simulink model "myo_sfun_one_myo_imu_emg"  (R2019a)
(part 8 of 12)

  "IW{2,1}(753,:)'" : Constant  Value=[0.783185612121389596040899050422012805938720703125;0.0661703247426442542344915409557870589196681976318359375;1.8359071026802709081238162980298511683940887451171875;-1.2946291113238352910030926068429835140705108642578125;-1.66363113612183166623026409070007503032684326171875;1.3769476811910852376286129583604633808135986328125;-0.82309788931886507246105111335054971277713775634765625;0.269452098677136542281829179046326316893100738525390625]
      mask Display: e = 0.06;c1 = [120 150 230]/255;c2 = ([120 150 230]+0)/383;c3 = ([120 150 230]+128)/383;patch([0 1 1 0],[0 0 1 1],c1);patch([0 1 1 1-e 1-e 0+e],[0 0 1 1-e 0+e 0+e],c2);patch([0 0 1 1-e 0+e 0+e],[0 1 1 1-e 1-e 0+e],c3);plot([0 1 1 0 0],[0 0 1 1 0]);disp('weights');
  "IW{2,1}(754,:)'" : Constant  Value=[-0.410530092885312336559167079030885361135005950927734375;-0.32543198628027558694242316050804220139980316162109375;0.257120581846906504086547329279710538685321807861328125;-1.4803527284791011542353089680545963346958160400390625;0.69265147232993451442695231889956630766391754150390625;1.1864451832958398114215015084482729434967041015625;2.49165954303533343505705488496460020542144775390625;-0.306699933021862436444138211300014518201351165771484375]
      mask Display: e = 0.06;c1 = [120 150 230]/255;c2 = ([120 150 230]+0)/383;c3 = ([120 150 230]+128)/383;patch([0 1 1 0],[0 0 1 1],c1);patch([0 1 1 1-e 1-e 0+e],[0 0 1 1-e 0+e 0+e],c2);patch([0 0 1 1-e 0+e 0+e],[0 1 1 1-e 1-e 0+e],c3);plot([0 1 1 0 0],[0 0 1 1 0]);disp('weights');
  "IW{2,1}(755,:)'" : Constant  Value=[-0.69971720416721427948658629247802309691905975341796875;0.379334814180492696511493022626382298767566680908203125;-1.66638817062355126807915439712814986705780029296875;-0.050359156796019884094750551639663171954452991485595703125;0.04393760587542960838192129813251085579395294189453125;-0.99442533329644466899566168649471364915370941162109375;-1.5735631371027520852834413744858466088771820068359375;2.045584518216794212008835529559291899204254150390625]
      mask Display: e = 0.06;c1 = [120 150 230]/255;c2 = ([120 150 230]+0)/383;c3 = ([120 150 230]+128)/383;patch([0 1 1 0],[0 0 1 1],c1);patch([0 1 1 1-e 1-e 0+e],[0 0 1 1-e 0+e 0+e],c2);patch([0 0 1 1-e 0+e 0+e],[0 1 1 1-e 1-e 0+e],c3);plot([0 1 1 0 0],[0 0 1 1 0]);disp('weights');
  "IW{2,1}(756,:)'" : Constant  Value=[1.8983314823386485681311341977561824023723602294921875;-1.6499514617594390752941535538411699235439300537109375;-1.592860658104178650518178983475081622600555419921875;-0.69510526567259212082916519648279063403606414794921875;-0.423661776374660348221112826649914495646953582763671875;0.302875746156102965134238047539838589727878570556640625;1.1171659130532229919907649673405103385448455810546875;-0.4960440878741383396999253818648867309093475341796875]
      mask Display: e = 0.06;c1 = [120 150 230]/255;c2 = ([120 150 230]+0)/383;c3 = ([120 150 230]+128)/383;patch([0 1 1 0],[0 0 1 1],c1);patch([0 1 1 1-e 1-e 0+e],[0 0 1 1-e 0+e 0+e],c2);patch([0 0 1 1-e 0+e 0+e],[0 1 1 1-e 1-e 0+e],c3);plot([0 1 1 0 0],[0 0 1 1 0]);disp('weights');
  "IW{2,1}(757,:)'" : Constant  Value=[1.5429828343096232412534618561039678752422332763671875;1.6031371671961582858756401037680916488170623779296875;0.1260080986217868292964539023159886710345745086669921875;-1.277218019145921257262443759827874600887298583984375;0.67625806402758803503871831708238460123538970947265625;0.308640418798115601095588544922065921127796173095703125;1.4325843178407087208370285225100815296173095703125;-1.352065283227812830801894961041398346424102783203125]
      mask Display: e = 0.06;c1 = [120 150 230]/255;c2 = ([120 150 230]+0)/383;c3 = ([120 150 230]+128)/383;patch([0 1 1 0],[0 0 1 1],c1);patch([0 1 1 1-e 1-e 0+e],[0 0 1 1-e 0+e 0+e],c2);patch([0 0 1 1-e 0+e 0+e],[0 1 1 1-e 1-e 0+e],c3);plot([0 1 1 0 0],[0 0 1 1 0]);disp('weights');
  "IW{2,1}(758,:)'" : Constant  Value=[-1.1493088977892480517795092964661307632923126220703125;0.198852045462145576859569473526789806783199310302734375;-0.97416051213436671840639746733359061181545257568359375;1.0286050667517485646129671295057050883769989013671875;-1.80797825924482413739724506740458309650421142578125;0.3406956718575855358466242250869981944561004638671875;1.834200275324268769594482364482246339321136474609375;-0.96161781439488447364993817245704121887683868408203125]
      mask Display: e = 0.06;c1 = [120 150 230]/255;c2 = ([120 150 230]+0)/383;c3 = ([120 150 230]+128)/383;patch([0 1 1 0],[0 0 1 1],c1);patch([0 1 1 1-e 1-e 0+e],[0 0 1 1-e 0+e 0+e],c2);patch([0 0 1 1-e 0+e 0+e],[0 1 1 1-e 1-e 0+e],c3);plot([0 1 1 0 0],[0 0 1 1 0]);disp('weights');
  "IW{2,1}(759,:)'" : Constant  Value=[1.3282172390572617448611936197266913950443267822265625;-1.6000852854439948647069513754104264080524444580078125;0.77939659454038190400382291045389138162136077880859375;1.1389255157510100868734070900245569646358489990234375;-0.0990875366675535163007992878192453645169734954833984375;1.6851010413502669482710416559712029993534088134765625;-7.354374628936846181904984920407741810777224600315093994140625e-05;1.40560043153014202488293449277989566326141357421875]
      mask Display: e = 0.06;c1 = [120 150 230]/255;c2 = ([120 150 230]+0)/383;c3 = ([120 150 230]+128)/383;patch([0 1 1 0],[0 0 1 1],c1);patch([0 1 1 1-e 1-e 0+e],[0 0 1 1-e 0+e 0+e],c2);patch([0 0 1 1-e 0+e 0+e],[0 1 1 1-e 1-e 0+e],c3);plot([0 1 1 0 0],[0 0 1 1 0]);disp('weights');
  "IW{2,1}(76,:)'" : Constant  Value=[1.5001171796290153626074470594176091253757476806640625;-1.5105423251143512697325377303059212863445281982421875;-0.1206347987803942645168575609204708598554134368896484375;1.0310345222403263232280323791201226413249969482421875;-0.47768382955221511121379762698779813945293426513671875;-1.3342813875335586271120291712577454745769500732421875;-1.6696874940304839984861473567434586584568023681640625;0.790028061013774873799775377847254276275634765625]
      mask Display: e = 0.06;c1 = [120 150 230]/255;c2 = ([120 150 230]+0)/383;c3 = ([120 150 230]+128)/383;patch([0 1 1 0],[0 0 1 1],c1);patch([0 1 1 1-e 1-e 0+e],[0 0 1 1-e 0+e 0+e],c2);patch([0 0 1 1-e 0+e 0+e],[0 1 1 1-e 1-e 0+e],c3);plot([0 1 1 0 0],[0 0 1 1 0]);disp('weights');
  "IW{2,1}(760,:)'" : Constant  Value=[-1.0176371041229881342360386042855679988861083984375;-1.872748358874109175786770720151253044605255126953125;-0.8315097219371649917007971453131176531314849853515625;0.82960320877955051610541659101727418601512908935546875;-0.7592772161929002283642375914496369659900665283203125;0.06569490608334704884185839546262286603450775146484375;1.6240039806704846814255915887770242989063262939453125;1.40670233447084580546970755676738917827606201171875]
      mask Display: e = 0.06;c1 = [120 150 230]/255;c2 = ([120 150 230]+0)/383;c3 = ([120 150 230]+128)/383;patch([0 1 1 0],[0 0 1 1],c1);patch([0 1 1 1-e 1-e 0+e],[0 0 1 1-e 0+e 0+e],c2);patch([0 0 1 1-e 0+e 0+e],[0 1 1 1-e 1-e 0+e],c3);plot([0 1 1 0 0],[0 0 1 1 0]);disp('weights');
  "IW{2,1}(761,:)'" : Constant  Value=[-1.4760895710418282522624622288276441395282745361328125;1.5449238983431639038457205970189534127712249755859375;-0.6414812240901774931245427069370634853839874267578125;1.228566998028169710011070492328144609928131103515625;-0.7253998641831866933671335573308169841766357421875;-0.477018391378114914314068073508678935468196868896484375;-1.72199388644027795436386440997011959552764892578125;0.8936550261419824447983728532562963664531707763671875]
      mask Display: e = 0.06;c1 = [120 150 230]/255;c2 = ([120 150 230]+0)/383;c3 = ([120 150 230]+128)/383;patch([0 1 1 0],[0 0 1 1],c1);patch([0 1 1 1-e 1-e 0+e],[0 0 1 1-e 0+e 0+e],c2);patch([0 0 1 1-e 0+e 0+e],[0 1 1 1-e 1-e 0+e],c3);plot([0 1 1 0 0],[0 0 1 1 0]);disp('weights');
  "IW{2,1}(762,:)'" : Constant  Value=[-1.40214953361763239314541351632215082645416259765625;0.0009893132168340671057926716258634769474156200885772705078125;-0.278198338550282586734141432316391728818416595458984375;-1.3089478916323198376403524889610707759857177734375;2.48707122269313796181222642189823091030120849609375;0.0655476063049824919648500554103520698845386505126953125;1.048706524249230387368925221380777657032012939453125;-0.61192488034971781463156048630480654537677764892578125]
      mask Display: e = 0.06;c1 = [120 150 230]/255;c2 = ([120 150 230]+0)/383;c3 = ([120 150 230]+128)/383;patch([0 1 1 0],[0 0 1 1],c1);patch([0 1 1 1-e 1-e 0+e],[0 0 1 1-e 0+e 0+e],c2);patch([0 0 1 1-e 0+e 0+e],[0 1 1 1-e 1-e 0+e],c3);plot([0 1 1 0 0],[0 0 1 1 0]);disp('weights');
  "IW{2,1}(763,:)'" : Constant  Value=[0.3202938735189400087932654059841297566890716552734375;2.180097427304347856846788999973796308040618896484375;0.6510959764016657214114047746988944709300994873046875;0.71099303337939112612531289414619095623493194580078125;2.27756408640566831991236540488898754119873046875;0.0237559841239538445389900545023920130915939807891845703125;0.12412617280098704741764237269308068789541721343994140625;0.1625160289190399065528680466741207055747509002685546875]
      mask Display: e = 0.06;c1 = [120 150 230]/255;c2 = ([120 150 230]+0)/383;c3 = ([120 150 230]+128)/383;patch([0 1 1 0],[0 0 1 1],c1);patch([0 1 1 1-e 1-e 0+e],[0 0 1 1-e 0+e 0+e],c2);patch([0 0 1 1-e 0+e 0+e],[0 1 1 1-e 1-e 0+e],c3);plot([0 1 1 0 0],[0 0 1 1 0]);disp('weights');
  "IW{2,1}(764,:)'" : Constant  Value=[-1.880922227720629447134115252993069589138031005859375;0.18169438580948515937762977046077139675617218017578125;-1.1208423860042591169161596553749404847621917724609375;0.82138794977296092358898249585763551294803619384765625;-0.445086336382885028317701880951062776148319244384765625;1.1356051656416890072165415404015220701694488525390625;1.53294095421436171733375886105932295322418212890625;1.3841953251573289040976533215143717825412750244140625]
      mask Display: e = 0.06;c1 = [120 150 230]/255;c2 = ([120 150 230]+0)/383;c3 = ([120 150 230]+128)/383;patch([0 1 1 0],[0 0 1 1],c1);patch([0 1 1 1-e 1-e 0+e],[0 0 1 1-e 0+e 0+e],c2);patch([0 0 1 1-e 0+e 0+e],[0 1 1 1-e 1-e 0+e],c3);plot([0 1 1 0 0],[0 0 1 1 0]);disp('weights');
  "IW{2,1}(765,:)'" : Constant  Value=[1.6480108777175477285936722182668745517730712890625;1.2350143728516480567947155577712692320346832275390625;-1.1626332226919344758897523206542246043682098388671875;-1.3273453269119546149568122928030788898468017578125;1.0338602880135654427107283481745980679988861083984375;0.82726662699471520401317548021324910223484039306640625;-0.868750821055978672546871166559867560863494873046875;-1.0568156825773098450582665464025922119617462158203125]
      mask Display: e = 0.06;c1 = [120 150 230]/255;c2 = ([120 150 230]+0)/383;c3 = ([120 150 230]+128)/383;patch([0 1 1 0],[0 0 1 1],c1);patch([0 1 1 1-e 1-e 0+e],[0 0 1 1-e 0+e 0+e],c2);patch([0 0 1 1-e 0+e 0+e],[0 1 1 1-e 1-e 0+e],c3);plot([0 1 1 0 0],[0 0 1 1 0]);disp('weights');
  "IW{2,1}(766,:)'" : Constant  Value=[0.2369511511416406979169124724649009294807910919189453125;-1.4120721645311677949763407013961113989353179931640625;0.37879224625033247608740794021287001669406890869140625;0.71627054433412185030505270333378575742244720458984375;-1.3351683021429676667679586898884736001491546630859375;1.5140182273159628056902192838606424629688262939453125;-1.08074438127618588367795382509939372539520263671875;1.8053836983539912619534106852370314300060272216796875]
      mask Display: e = 0.06;c1 = [120 150 230]/255;c2 = ([120 150 230]+0)/383;c3 = ([120 150 230]+128)/383;patch([0 1 1 0],[0 0 1 1],c1);patch([0 1 1 1-e 1-e 0+e],[0 0 1 1-e 0+e 0+e],c2);patch([0 0 1 1-e 0+e 0+e],[0 1 1 1-e 1-e 0+e],c3);plot([0 1 1 0 0],[0 0 1 1 0]);disp('weights');
  "IW{2,1}(767,:)'" : Constant  Value=[0.0010137896241931803990865557096867632935754954814910888671875;-1.739136278505398980342988579650409519672393798828125;0.12339190484929184188356288132126792334020137786865234375;-1.68026618448033548958164828945882618427276611328125;0.9238204519764057209840757423080503940582275390625;-0.1157783217733323322118366149879875592887401580810546875;1.4456548668953030922779134925804100930690765380859375;1.5122354198140659509164152041194029152393341064453125]
      mask Display: e = 0.06;c1 = [120 150 230]/255;c2 = ([120 150 230]+0)/383;c3 = ([120 150 230]+128)/383;patch([0 1 1 0],[0 0 1 1],c1);patch([0 1 1 1-e 1-e 0+e],[0 0 1 1-e 0+e 0+e],c2);patch([0 0 1 1-e 0+e 0+e],[0 1 1 1-e 1-e 0+e],c3);plot([0 1 1 0 0],[0 0 1 1 0]);disp('weights');
  "IW{2,1}(768,:)'" : Constant  Value=[0.57912060665102649270608026199624873697757720947265625;-0.3015274233909204237846779506071470677852630615234375;0.1761144065427179550287206666325801052153110504150390625;0.481347550919307476391395539394579827785491943359375;-0.826138806546137249853245521080680191516876220703125;2.852716196456658526159344546613283455371856689453125;-1.2339068046680565782224903159658424556255340576171875;0.0028978835039482060513538197454863620805554091930389404296875]
      mask Display: e = 0.06;c1 = [120 150 230]/255;c2 = ([120 150 230]+0)/383;c3 = ([120 150 230]+128)/383;patch([0 1 1 0],[0 0 1 1],c1);patch([0 1 1 1-e 1-e 0+e],[0 0 1 1-e 0+e 0+e],c2);patch([0 0 1 1-e 0+e 0+e],[0 1 1 1-e 1-e 0+e],c3);plot([0 1 1 0 0],[0 0 1 1 0]);disp('weights');
  "IW{2,1}(769,:)'" : Constant  Value=[0.78586784355456751338664389550103805959224700927734375;0.5155840752440845609072539446060545742511749267578125;-1.4603002716642665692603486604639329016208648681640625;-1.59285262440896335789375370950438082218170166015625;-1.46770658790118257996937245479784905910491943359375;1.213265132572129090249291039071977138519287109375;-0.98696981478665379849957162150531075894832611083984375;-1.1179206552264304708188547010649926960468292236328125]
      mask Display: e = 0.06;c1 = [120 150 230]/255;c2 = ([120 150 230]+0)/383;c3 = ([120 150 230]+128)/383;patch([0 1 1 0],[0 0 1 1],c1);patch([0 1 1 1-e 1-e 0+e],[0 0 1 1-e 0+e 0+e],c2);patch([0 0 1 1-e 0+e 0+e],[0 1 1 1-e 1-e 0+e],c3);plot([0 1 1 0 0],[0 0 1 1 0]);disp('weights');
  "IW{2,1}(77,:)'" : Constant  Value=[0.94967604944117345322496248627430759370326995849609375;-1.5403680775541050973487244846182875335216522216796875;1.5908176635751611893709878131630830466747283935546875;-0.5311955915482473589150913539924658834934234619140625;-1.1887843111091120906763762832270003855228424072265625;-1.0854926151946437951067991889431141316890716552734375;0.423786694687962650629486915931920520961284637451171875;1.466556061921565845551640450139530003070831298828125]
      mask Display: e = 0.06;c1 = [120 150 230]/255;c2 = ([120 150 230]+0)/383;c3 = ([120 150 230]+128)/383;patch([0 1 1 0],[0 0 1 1],c1);patch([0 1 1 1-e 1-e 0+e],[0 0 1 1-e 0+e 0+e],c2);patch([0 0 1 1-e 0+e 0+e],[0 1 1 1-e 1-e 0+e],c3);plot([0 1 1 0 0],[0 0 1 1 0]);disp('weights');
  "IW{2,1}(770,:)'" : Constant  Value=[-1.60309206066617715435995705774985253810882568359375;-0.51783532205714533080964656619471497833728790283203125;-1.2924390595397614589501245063729584217071533203125;-0.47354576106205537033844166217022575438022613525390625;-1.231551733349906641024062992073595523834228515625;1.282123209632743954244915585150010883808135986328125;-1.339041605027291748086781808524392545223236083984375;1.158346776423092361341105061001144349575042724609375]
      mask Display: e = 0.06;c1 = [120 150 230]/255;c2 = ([120 150 230]+0)/383;c3 = ([120 150 230]+128)/383;patch([0 1 1 0],[0 0 1 1],c1);patch([0 1 1 1-e 1-e 0+e],[0 0 1 1-e 0+e 0+e],c2);patch([0 0 1 1-e 0+e 0+e],[0 1 1 1-e 1-e 0+e],c3);plot([0 1 1 0 0],[0 0 1 1 0]);disp('weights');
  "IW{2,1}(771,:)'" : Constant  Value=[-0.10844966992756878421122479494442814029753208160400390625;-2.04097879690192485213628970086574554443359375;-1.8467790540451012315514844885910861194133758544921875;-0.304314585816960303521483410804648883640766143798828125;0.265009741844671686816781175366486422717571258544921875;0.6898099317531134477832210905035026371479034423828125;1.0382473016672901788837179992697201669216156005859375;-1.3107954550942937377300268053659237921237945556640625]
      mask Display: e = 0.06;c1 = [120 150 230]/255;c2 = ([120 150 230]+0)/383;c3 = ([120 150 230]+128)/383;patch([0 1 1 0],[0 0 1 1],c1);patch([0 1 1 1-e 1-e 0+e],[0 0 1 1-e 0+e 0+e],c2);patch([0 0 1 1-e 0+e 0+e],[0 1 1 1-e 1-e 0+e],c3);plot([0 1 1 0 0],[0 0 1 1 0]);disp('weights');
  "IW{2,1}(772,:)'" : Constant  Value=[-1.517050479000064289181182175525464117527008056640625;1.3725659899028095356499079571221955120563507080078125;1.0270065742732679137105833433452062308788299560546875;-0.93487453061604097737102847531787119805812835693359375;0.68189963435994283003083182848058640956878662109375;-1.4158641006984373778010422029183246195316314697265625;-1.5124736179747910735926552661112509667873382568359375;-0.38433165867158403106174091590219177305698394775390625]
      mask Display: e = 0.06;c1 = [120 150 230]/255;c2 = ([120 150 230]+0)/383;c3 = ([120 150 230]+128)/383;patch([0 1 1 0],[0 0 1 1],c1);patch([0 1 1 1-e 1-e 0+e],[0 0 1 1-e 0+e 0+e],c2);patch([0 0 1 1-e 0+e 0+e],[0 1 1 1-e 1-e 0+e],c3);plot([0 1 1 0 0],[0 0 1 1 0]);disp('weights');
  "IW{2,1}(773,:)'" : Constant  Value=[-1.259219760630129858469672399223782122135162353515625;0.40369571030896123087217119973502121865749359130859375;-1.45176564970109467367365141399204730987548828125;-0.590275130419540605686279377550818026065826416015625;0.6519510871785050287741114516393281519412994384765625;-1.7422522773703554843649499161983840167522430419921875;1.80382679092467324011295204400084912776947021484375;-0.337580493884244325908383643763954751193523406982421875]
      mask Display: e = 0.06;c1 = [120 150 230]/255;c2 = ([120 150 230]+0)/383;c3 = ([120 150 230]+128)/383;patch([0 1 1 0],[0 0 1 1],c1);patch([0 1 1 1-e 1-e 0+e],[0 0 1 1-e 0+e 0+e],c2);patch([0 0 1 1-e 0+e 0+e],[0 1 1 1-e 1-e 0+e],c3);plot([0 1 1 0 0],[0 0 1 1 0]);disp('weights');
  "IW{2,1}(774,:)'" : Constant  Value=[1.0494588447924539931221943334094248712062835693359375;2.2426691579786588448541806428693234920501708984375;-0.3960160180596938861441458357148803770542144775390625;-0.2418699441399993765866582862145151011645793914794921875;0.295309949651697156713936465166625566780567169189453125;0.37702138534180573703480376934749074280261993408203125;0.386653205873825289717871100947377271950244903564453125;-2.0733438359517943894161362550221383571624755859375]
      mask Display: e = 0.06;c1 = [120 150 230]/255;c2 = ([120 150 230]+0)/383;c3 = ([120 150 230]+128)/383;patch([0 1 1 0],[0 0 1 1],c1);patch([0 1 1 1-e 1-e 0+e],[0 0 1 1-e 0+e 0+e],c2);patch([0 0 1 1-e 0+e 0+e],[0 1 1 1-e 1-e 0+e],c3);plot([0 1 1 0 0],[0 0 1 1 0]);disp('weights');
  "IW{2,1}(775,:)'" : Constant  Value=[1.002703173940568515121185555472038686275482177734375;-0.454218764977076860933635771289118565618991851806640625;0.2247979254728177112010456539792357943952083587646484375;0.95350044750633167200959405818139202892780303955078125;1.497138541129345856717236529220826923847198486328125;1.8020649003205033711338955981773324310779571533203125;-0.55227649259595057440463961029308848083019256591796875;-1.7603145213687529935242537248996086418628692626953125]
      mask Display: e = 0.06;c1 = [120 150 230]/255;c2 = ([120 150 230]+0)/383;c3 = ([120 150 230]+128)/383;patch([0 1 1 0],[0 0 1 1],c1);patch([0 1 1 1-e 1-e 0+e],[0 0 1 1-e 0+e 0+e],c2);patch([0 0 1 1-e 0+e 0+e],[0 1 1 1-e 1-e 0+e],c3);plot([0 1 1 0 0],[0 0 1 1 0]);disp('weights');
  "IW{2,1}(776,:)'" : Constant  Value=[-1.22814884809633184659105609171092510223388671875;-1.0010532688682953761372118606232106685638427734375;-0.97817402122436092337665058948914520442485809326171875;-1.2737862865739355555660949903540313243865966796875;1.56447940989051659244069014675915241241455078125;1.4241609039559197658064704228308983147144317626953125;1.3307174274438879901794052784680388867855072021484375;-0.054111943261800306281816830278330598957836627960205078125]
      mask Display: e = 0.06;c1 = [120 150 230]/255;c2 = ([120 150 230]+0)/383;c3 = ([120 150 230]+128)/383;patch([0 1 1 0],[0 0 1 1],c1);patch([0 1 1 1-e 1-e 0+e],[0 0 1 1-e 0+e 0+e],c2);patch([0 0 1 1-e 0+e 0+e],[0 1 1 1-e 1-e 0+e],c3);plot([0 1 1 0 0],[0 0 1 1 0]);disp('weights');
  "IW{2,1}(777,:)'" : Constant  Value=[-1.6705477679523121903315541203483007848262786865234375;-0.50565751089381161254010521588497795164585113525390625;0.374129381175553221705598616608767770230770111083984375;1.24140950769124014385624832357279956340789794921875;1.270901094959212773716217270703054964542388916015625;1.5702246279509715076727616178686730563640594482421875;-0.66101625344364511871475542648113332688808441162109375;1.3563305258847850875980611817794851958751678466796875]
      mask Display: e = 0.06;c1 = [120 150 230]/255;c2 = ([120 150 230]+0)/383;c3 = ([120 150 230]+128)/383;patch([0 1 1 0],[0 0 1 1],c1);patch([0 1 1 1-e 1-e 0+e],[0 0 1 1-e 0+e 0+e],c2);patch([0 0 1 1-e 0+e 0+e],[0 1 1 1-e 1-e 0+e],c3);plot([0 1 1 0 0],[0 0 1 1 0]);disp('weights');
  "IW{2,1}(778,:)'" : Constant  Value=[1.35356910036644517703052770229987800121307373046875;0.477217492069804849474934371755807660520076751708984375;-1.462099461724876814372464650659821927547454833984375;0.247249741115579457773065996661898680031299591064453125;-1.157008536204823911930361646227538585662841796875;-1.55515736444071261956878515775315463542938232421875;0.451936526566375729174751540995202958583831787109375;1.6690619145797871425429548253305256366729736328125]
      mask Display: e = 0.06;c1 = [120 150 230]/255;c2 = ([120 150 230]+0)/383;c3 = ([120 150 230]+128)/383;patch([0 1 1 0],[0 0 1 1],c1);patch([0 1 1 1-e 1-e 0+e],[0 0 1 1-e 0+e 0+e],c2);patch([0 0 1 1-e 0+e 0+e],[0 1 1 1-e 1-e 0+e],c3);plot([0 1 1 0 0],[0 0 1 1 0]);disp('weights');
  "IW{2,1}(779,:)'" : Constant  Value=[-0.65572414623703323410808252447168342769145965576171875;-1.47638054734529422518107821815647184848785400390625;1.4200021275675940302107846946455538272857666015625;-0.30664106971060156592301382261211983859539031982421875;-1.170123515920813428436986214364878833293914794921875;1.0749549288145419101425659391679801046848297119140625;-1.16104467805839117744426403078250586986541748046875;-1.5631502570277360231187913086614571511745452880859375]
      mask Display: e = 0.06;c1 = [120 150 230]/255;c2 = ([120 150 230]+0)/383;c3 = ([120 150 230]+128)/383;patch([0 1 1 0],[0 0 1 1],c1);patch([0 1 1 1-e 1-e 0+e],[0 0 1 1-e 0+e 0+e],c2);patch([0 0 1 1-e 0+e 0+e],[0 1 1 1-e 1-e 0+e],c3);plot([0 1 1 0 0],[0 0 1 1 0]);disp('weights');
  "IW{2,1}(78,:)'" : Constant  Value=[-0.1407466047710739243115085628232918679714202880859375;0.73016064899796095932771322623011656105518341064453125;1.8139492608273080076486394318635575473308563232421875;-1.945663194925956407388412117143161594867706298828125;0.0617384857237628092985204375509056262671947479248046875;-0.56428916929213090991623857917147688567638397216796875;-1.5004695410340704864182725941645912826061248779296875;0.82762841741629900038645928361802361905574798583984375]
      mask Display: e = 0.06;c1 = [120 150 230]/255;c2 = ([120 150 230]+0)/383;c3 = ([120 150 230]+128)/383;patch([0 1 1 0],[0 0 1 1],c1);patch([0 1 1 1-e 1-e 0+e],[0 0 1 1-e 0+e 0+e],c2);patch([0 0 1 1-e 0+e 0+e],[0 1 1 1-e 1-e 0+e],c3);plot([0 1 1 0 0],[0 0 1 1 0]);disp('weights');
  "IW{2,1}(780,:)'" : Constant  Value=[1.20472405892639766733509532059542834758758544921875;-2.177781407949598957429770962335169315338134765625;0.879613284465513789456281301681883633136749267578125;0.5214726388915311705574140432872809469699859619140625;1.8957001374363715573423405658104456961154937744140625;-0.31560867712000117979442848081816919147968292236328125;-0.2234332478380625930380887211867957375943660736083984375;-0.193737563261967171701627421498415060341358184814453125]
      mask Display: e = 0.06;c1 = [120 150 230]/255;c2 = ([120 150 230]+0)/383;c3 = ([120 150 230]+128)/383;patch([0 1 1 0],[0 0 1 1],c1);patch([0 1 1 1-e 1-e 0+e],[0 0 1 1-e 0+e 0+e],c2);patch([0 0 1 1-e 0+e 0+e],[0 1 1 1-e 1-e 0+e],c3);plot([0 1 1 0 0],[0 0 1 1 0]);disp('weights');
  "IW{2,1}(781,:)'" : Constant  Value=[2.76122829079074971758700485224835574626922607421875;-1.0623002987083018933134326289291493594646453857421875;0.1207554539788972813862955035801860503852367401123046875;-0.307599399992625588406980341460439376533031463623046875;-0.392854501898636687684529533726163208484649658203125;0.5738833622648069621163813280873000621795654296875;-1.3719460130582936674414895605877973139286041259765625;-0.05634072474674400865524148684926331043243408203125]
      mask Display: e = 0.06;c1 = [120 150 230]/255;c2 = ([120 150 230]+0)/383;c3 = ([120 150 230]+128)/383;patch([0 1 1 0],[0 0 1 1],c1);patch([0 1 1 1-e 1-e 0+e],[0 0 1 1-e 0+e 0+e],c2);patch([0 0 1 1-e 0+e 0+e],[0 1 1 1-e 1-e 0+e],c3);plot([0 1 1 0 0],[0 0 1 1 0]);disp('weights');
  "IW{2,1}(782,:)'" : Constant  Value=[-1.9322641936651330230034773194347508251667022705078125;-1.00629887395713968345489774947054684162139892578125;1.7747060806392889187321770805283449590206146240234375;0.49385409080588671404399292441667057573795318603515625;0.7713497590596443131971682305447757244110107421875;-0.130146787075340053529970418821903876960277557373046875;1.3509523785146477781182738908682949841022491455078125;0.6259672295324729685006559520843438804149627685546875]
      mask Display: e = 0.06;c1 = [120 150 230]/255;c2 = ([120 150 230]+0)/383;c3 = ([120 150 230]+128)/383;patch([0 1 1 0],[0 0 1 1],c1);patch([0 1 1 1-e 1-e 0+e],[0 0 1 1-e 0+e 0+e],c2);patch([0 0 1 1-e 0+e 0+e],[0 1 1 1-e 1-e 0+e],c3);plot([0 1 1 0 0],[0 0 1 1 0]);disp('weights');
  "IW{2,1}(783,:)'" : Constant  Value=[1.6893988429284172436695143915130756795406341552734375;0.225913592569459253933672471248428337275981903076171875;-1.243388397209162832268702914007008075714111328125;-1.862060440104080338841185948695056140422821044921875;-0.2447434177893425266692162267645471729338169097900390625;1.3641230092016243258257190973381511867046356201171875;-0.207361012426501900574038472768734209239482879638671875;-1.0513234460344680343268919386900961399078369140625]
      mask Display: e = 0.06;c1 = [120 150 230]/255;c2 = ([120 150 230]+0)/383;c3 = ([120 150 230]+128)/383;patch([0 1 1 0],[0 0 1 1],c1);patch([0 1 1 1-e 1-e 0+e],[0 0 1 1-e 0+e 0+e],c2);patch([0 0 1 1-e 0+e 0+e],[0 1 1 1-e 1-e 0+e],c3);plot([0 1 1 0 0],[0 0 1 1 0]);disp('weights');
  "IW{2,1}(784,:)'" : Constant  Value=[1.0620272474208132251760616782121360301971435546875;0.47233971658456874731513153164996765553951263427734375;-0.172945943348280339879607936381944455206394195556640625;-1.506887071281265644273616999271325767040252685546875;1.7618509452182180563539759532432071864604949951171875;-0.5532461673119841716328437541960738599300384521484375;1.2244093360544543447332443975028581917285919189453125;-1.56237266831900978303337979014031589031219482421875]
      mask Display: e = 0.06;c1 = [120 150 230]/255;c2 = ([120 150 230]+0)/383;c3 = ([120 150 230]+128)/383;patch([0 1 1 0],[0 0 1 1],c1);patch([0 1 1 1-e 1-e 0+e],[0 0 1 1-e 0+e 0+e],c2);patch([0 0 1 1-e 0+e 0+e],[0 1 1 1-e 1-e 0+e],c3);plot([0 1 1 0 0],[0 0 1 1 0]);disp('weights');
  "IW{2,1}(785,:)'" : Constant  Value=[-0.179395783995652979836421536674606613814830780029296875;-1.6818566757074220330281377755454741418361663818359375;0.09648496457834822292998211423764587379992008209228515625;0.1518050950382008046357640296264435164630413055419921875;-0.03010888320754999403217055942150182090699672698974609375;-2.298440485049809023365696702967397868633270263671875;-1.5154241120918168217457377977552823722362518310546875;0.74505564941249524668620551892672665417194366455078125]
      mask Display: e = 0.06;c1 = [120 150 230]/255;c2 = ([120 150 230]+0)/383;c3 = ([120 150 230]+128)/383;patch([0 1 1 0],[0 0 1 1],c1);patch([0 1 1 1-e 1-e 0+e],[0 0 1 1-e 0+e 0+e],c2);patch([0 0 1 1-e 0+e 0+e],[0 1 1 1-e 1-e 0+e],c3);plot([0 1 1 0 0],[0 0 1 1 0]);disp('weights');
  "IW{2,1}(786,:)'" : Constant  Value=[-1.3425414948095168998776216540136374533176422119140625;-0.0890896214824471732729449513499275781214237213134765625;1.724918800885346659157448812038637697696685791015625;-0.10471661262302543737856552752418792806565761566162109375;0.5625814408031770685880701421410776674747467041015625;0.42245581594058012608883245775359682738780975341796875;-1.2459249951450239723982349460129626095294952392578125;-2.03035397967017150477886389126069843769073486328125]
      mask Display: e = 0.06;c1 = [120 150 230]/255;c2 = ([120 150 230]+0)/383;c3 = ([120 150 230]+128)/383;patch([0 1 1 0],[0 0 1 1],c1);patch([0 1 1 1-e 1-e 0+e],[0 0 1 1-e 0+e 0+e],c2);patch([0 0 1 1-e 0+e 0+e],[0 1 1 1-e 1-e 0+e],c3);plot([0 1 1 0 0],[0 0 1 1 0]);disp('weights');
  "IW{2,1}(787,:)'" : Constant  Value=[1.0854688131216720936578212786116637289524078369140625;1.786746059171278933064286320586688816547393798828125;0.12200539984674622917548703071588533930480480194091796875;-0.81146003915904285630489312097779475152492523193359375;0.5279805453242392143664574177819304168224334716796875;0.90394730071178852615076948495698161423206329345703125;-1.448571074143185644089726338279433548450469970703125;-1.6602820646698066564539431055891327559947967529296875]
      mask Display: e = 0.06;c1 = [120 150 230]/255;c2 = ([120 150 230]+0)/383;c3 = ([120 150 230]+128)/383;patch([0 1 1 0],[0 0 1 1],c1);patch([0 1 1 1-e 1-e 0+e],[0 0 1 1-e 0+e 0+e],c2);patch([0 0 1 1-e 0+e 0+e],[0 1 1 1-e 1-e 0+e],c3);plot([0 1 1 0 0],[0 0 1 1 0]);disp('weights');
  "IW{2,1}(788,:)'" : Constant  Value=[-0.4698990953664019531998974343878217041492462158203125;2.228625086753846407106038896017707884311676025390625;0.97039922697363512060775292411562986671924591064453125;1.18753777081516975755448584095574915409088134765625;-1.2771933791042002770410590528626926243305206298828125;-0.19264632613096621671644470552564598619937896728515625;-0.6946821823975983800636413434403948485851287841796875;-1.1048478483617836243269039186998270452022552490234375]
      mask Display: e = 0.06;c1 = [120 150 230]/255;c2 = ([120 150 230]+0)/383;c3 = ([120 150 230]+128)/383;patch([0 1 1 0],[0 0 1 1],c1);patch([0 1 1 1-e 1-e 0+e],[0 0 1 1-e 0+e 0+e],c2);patch([0 0 1 1-e 0+e 0+e],[0 1 1 1-e 1-e 0+e],c3);plot([0 1 1 0 0],[0 0 1 1 0]);disp('weights');
  "IW{2,1}(789,:)'" : Constant  Value=[-1.1954349322313342351975506971939466893672943115234375;0.254954615905215342674949852153076790273189544677734375;-0.729027390173369926884561209590174257755279541015625;-1.2801448826580050788237485903664492070674896240234375;1.7653475584719651170217957769636996090412139892578125;1.273154332788164477818781961104832589626312255859375;0.297162851983625297958013788957032375037670135498046875;1.607461357218479491848484030924737453460693359375]
      mask Display: e = 0.06;c1 = [120 150 230]/255;c2 = ([120 150 230]+0)/383;c3 = ([120 150 230]+128)/383;patch([0 1 1 0],[0 0 1 1],c1);patch([0 1 1 1-e 1-e 0+e],[0 0 1 1-e 0+e 0+e],c2);patch([0 0 1 1-e 0+e 0+e],[0 1 1 1-e 1-e 0+e],c3);plot([0 1 1 0 0],[0 0 1 1 0]);disp('weights');
  "IW{2,1}(79,:)'" : Constant  Value=[-1.454345653793586823354644366190768778324127197265625;-1.5000053456295894260819068222190253436565399169921875;-0.1190879144108819287506406681131920777261257171630859375;0.01259612237224565743642923365541719249449670314788818359375;1.4220388141981465945917761928285472095012664794921875;-0.350444949810018446800796709794667549431324005126953125;-1.4862134480305819739243133881245739758014678955078125;1.6082221761231014767190572456456720829010009765625]
      mask Display: e = 0.06;c1 = [120 150 230]/255;c2 = ([120 150 230]+0)/383;c3 = ([120 150 230]+128)/383;patch([0 1 1 0],[0 0 1 1],c1);patch([0 1 1 1-e 1-e 0+e],[0 0 1 1-e 0+e 0+e],c2);patch([0 0 1 1-e 0+e 0+e],[0 1 1 1-e 1-e 0+e],c3);plot([0 1 1 0 0],[0 0 1 1 0]);disp('weights');
  "IW{2,1}(790,:)'" : Constant  Value=[-0.3499584335750405283960162705625407397747039794921875;1.4123167729368490963537396964966319501399993896484375;1.0513137201449305191403027492924593389034271240234375;-1.6753309471439685740534741853480227291584014892578125;-0.143085928295401398901987022327375598251819610595703125;0.9409164128731362097823875956237316131591796875;-1.2519447014244640126179319850052706897258758544921875;-1.66698599786439505265889238216914236545562744140625]
      mask Display: e = 0.06;c1 = [120 150 230]/255;c2 = ([120 150 230]+0)/383;c3 = ([120 150 230]+128)/383;patch([0 1 1 0],[0 0 1 1],c1);patch([0 1 1 1-e 1-e 0+e],[0 0 1 1-e 0+e 0+e],c2);patch([0 0 1 1-e 0+e 0+e],[0 1 1 1-e 1-e 0+e],c3);plot([0 1 1 0 0],[0 0 1 1 0]);disp('weights');
  "IW{2,1}(791,:)'" : Constant  Value=[-1.6212226087080814362906266978825442492961883544921875;-0.00664598725078462647386512429648064426146447658538818359375;-0.497774706925136645185858697004732675850391387939453125;-0.8965190674538294768325386030483059585094451904296875;1.8128340585994402456293528302921913564205169677734375;-0.251152548948948839413475297988043166697025299072265625;0.11213514945235657227495806864681071601808071136474609375;-1.9991787235258726695974473841488361358642578125]
      mask Display: e = 0.06;c1 = [120 150 230]/255;c2 = ([120 150 230]+0)/383;c3 = ([120 150 230]+128)/383;patch([0 1 1 0],[0 0 1 1],c1);patch([0 1 1 1-e 1-e 0+e],[0 0 1 1-e 0+e 0+e],c2);patch([0 0 1 1-e 0+e 0+e],[0 1 1 1-e 1-e 0+e],c3);plot([0 1 1 0 0],[0 0 1 1 0]);disp('weights');
  "IW{2,1}(792,:)'" : Constant  Value=[-1.6602606604656544586617883396684192121028900146484375;-0.8496114760869364346262955223210155963897705078125;-0.35104782957804758769526642936398275196552276611328125;-1.656826004383271655484577422612346708774566650390625;-1.4346878897252810514117982165771536529064178466796875;0.165466029757858124060732052384992130100727081298828125;1.5734664279879722048605117379338480532169342041015625;0.337872835146016570195826034250785596668720245361328125]
      mask Display: e = 0.06;c1 = [120 150 230]/255;c2 = ([120 150 230]+0)/383;c3 = ([120 150 230]+128)/383;patch([0 1 1 0],[0 0 1 1],c1);patch([0 1 1 1-e 1-e 0+e],[0 0 1 1-e 0+e 0+e],c2);patch([0 0 1 1-e 0+e 0+e],[0 1 1 1-e 1-e 0+e],c3);plot([0 1 1 0 0],[0 0 1 1 0]);disp('weights');
  "IW{2,1}(793,:)'" : Constant  Value=[0.1354401986727943596466872122618951834738254547119140625;1.4280561271352458785344197167432866990566253662109375;-1.87261754727813212184628355316817760467529296875;-0.94910855722564801961738112368038855493068695068359375;-1.1031033185725658274378702117246575653553009033203125;-0.0222369875416463837203284725774210528470575809478759765625;-0.1605962650882052089595930510768084786832332611083984375;-1.7818971070551381519209144244086928665637969970703125]
      mask Display: e = 0.06;c1 = [120 150 230]/255;c2 = ([120 150 230]+0)/383;c3 = ([120 150 230]+128)/383;patch([0 1 1 0],[0 0 1 1],c1);patch([0 1 1 1-e 1-e 0+e],[0 0 1 1-e 0+e 0+e],c2);patch([0 0 1 1-e 0+e 0+e],[0 1 1 1-e 1-e 0+e],c3);plot([0 1 1 0 0],[0 0 1 1 0]);disp('weights');
  "IW{2,1}(794,:)'" : Constant  Value=[-0.0960306740130501823582420684033422730863094329833984375;0.8638031410457929215596095673390664160251617431640625;-1.96871235086645501866087215603329241275787353515625;1.7314153981485873590173696356941945850849151611328125;0.1530734069582344869520085239855688996613025665283203125;-0.440234092943701416089652411756105720996856689453125;1.1041120436467135590419275104068219661712646484375;-1.3741051332568099407893669194891117513179779052734375]
      mask Display: e = 0.06;c1 = [120 150 230]/255;c2 = ([120 150 230]+0)/383;c3 = ([120 150 230]+128)/383;patch([0 1 1 0],[0 0 1 1],c1);patch([0 1 1 1-e 1-e 0+e],[0 0 1 1-e 0+e 0+e],c2);patch([0 0 1 1-e 0+e 0+e],[0 1 1 1-e 1-e 0+e],c3);plot([0 1 1 0 0],[0 0 1 1 0]);disp('weights');
  "IW{2,1}(795,:)'" : Constant  Value=[-1.74714618328577131478596129454672336578369140625;1.4846747087115963470438373406068421900272369384765625;1.07823301920891623240095213986933231353759765625;-1.379851251816174961817296207300387322902679443359375;0.069145191657301430243620643523172475397586822509765625;-0.9033876654740475853344605638994835317134857177734375;-1.3328426873114216366644768640981055796146392822265625;-0.311923707529923321946085934541770257055759429931640625]
      mask Display: e = 0.06;c1 = [120 150 230]/255;c2 = ([120 150 230]+0)/383;c3 = ([120 150 230]+128)/383;patch([0 1 1 0],[0 0 1 1],c1);patch([0 1 1 1-e 1-e 0+e],[0 0 1 1-e 0+e 0+e],c2);patch([0 0 1 1-e 0+e 0+e],[0 1 1 1-e 1-e 0+e],c3);plot([0 1 1 0 0],[0 0 1 1 0]);disp('weights');
  "IW{2,1}(796,:)'" : Constant  Value=[1.5360295984492624565831420113681815564632415771484375;-1.7131536346822178185078655587858520448207855224609375;1.5768894968390656519119374934234656393527984619140625;0.173944353712400745504140786579228006303310394287109375;0.79084525076776934771061178253148682415485382080078125;-1.5519147608880408117926208433345891535282135009765625;0.449312404307729895691636556875891983509063720703125;0.2008602463838435603360466075173462741076946258544921875]
      mask Display: e = 0.06;c1 = [120 150 230]/255;c2 = ([120 150 230]+0)/383;c3 = ([120 150 230]+128)/383;patch([0 1 1 0],[0 0 1 1],c1);patch([0 1 1 1-e 1-e 0+e],[0 0 1 1-e 0+e 0+e],c2);patch([0 0 1 1-e 0+e 0+e],[0 1 1 1-e 1-e 0+e],c3);plot([0 1 1 0 0],[0 0 1 1 0]);disp('weights');
  "IW{2,1}(797,:)'" : Constant  Value=[-1.495008703605724686980238402611576020717620849609375;1.9677376501445831280534548568539321422576904296875;-0.8889135426196619338412574506946839392185211181640625;-0.68873017130275016040030777730862610042095184326171875;0.01846611302918534092132318846779526211321353912353515625;-0.90698722045707336203435033894493244588375091552734375;0.386944048199925505482354992636828683316707611083984375;-1.628627614236950904569312115199863910675048828125]
      mask Display: e = 0.06;c1 = [120 150 230]/255;c2 = ([120 150 230]+0)/383;c3 = ([120 150 230]+128)/383;patch([0 1 1 0],[0 0 1 1],c1);patch([0 1 1 1-e 1-e 0+e],[0 0 1 1-e 0+e 0+e],c2);patch([0 0 1 1-e 0+e 0+e],[0 1 1 1-e 1-e 0+e],c3);plot([0 1 1 0 0],[0 0 1 1 0]);disp('weights');
  "IW{2,1}(798,:)'" : Constant  Value=[1.596004342975323897491080060717649757862091064453125;0.0640950793087518289059545395502937026321887969970703125;0.6741903079137110399443599817459471523761749267578125;0.48545664911829355947503472634707577526569366455078125;1.4778553222691892532481006128364242613315582275390625;-1.9975412567322836654426509994664229452610015869140625;-0.273894928528651104837621232945821247994899749755859375;-1.2236279018843436716679207165725529193878173828125]
      mask Display: e = 0.06;c1 = [120 150 230]/255;c2 = ([120 150 230]+0)/383;c3 = ([120 150 230]+128)/383;patch([0 1 1 0],[0 0 1 1],c1);patch([0 1 1 1-e 1-e 0+e],[0 0 1 1-e 0+e 0+e],c2);patch([0 0 1 1-e 0+e 0+e],[0 1 1 1-e 1-e 0+e],c3);plot([0 1 1 0 0],[0 0 1 1 0]);disp('weights');
  "IW{2,1}(799,:)'" : Constant  Value=[1.4770375632864567450042159180156886577606201171875;0.693385839689065530677680726512335240840911865234375;-0.71747562482047311238630982188624329864978790283203125;0.5514079574493659929856903545442037284374237060546875;1.537506493843416865985318509046919643878936767578125;0.79357515376455667333033261456876061856746673583984375;-1.76544500847806862253719373256899416446685791015625;1.1878881439392756647066562436521053314208984375]
      mask Display: e = 0.06;c1 = [120 150 230]/255;c2 = ([120 150 230]+0)/383;c3 = ([120 150 230]+128)/383;patch([0 1 1 0],[0 0 1 1],c1);patch([0 1 1 1-e 1-e 0+e],[0 0 1 1-e 0+e 0+e],c2);patch([0 0 1 1-e 0+e 0+e],[0 1 1 1-e 1-e 0+e],c3);plot([0 1 1 0 0],[0 0 1 1 0]);disp('weights');
  "IW{2,1}(8,:)'" : Constant  Value=[1.6190915800654364087307612862787209451198577880859375;-1.002926456833790336276024390826933085918426513671875;-1.343600877266364790330044343136250972747802734375;0.92353566004879483752887381342588923871517181396484375;-1.18433082284919510840381917660124599933624267578125;0.317507488243029711849629848074982874095439910888671875;-1.7946898445228784968463742188760079443454742431640625;-0.0787404021836220768815195469869649969041347503662109375]
      mask Display: e = 0.06;c1 = [120 150 230]/255;c2 = ([120 150 230]+0)/383;c3 = ([120 150 230]+128)/383;patch([0 1 1 0],[0 0 1 1],c1);patch([0 1 1 1-e 1-e 0+e],[0 0 1 1-e 0+e 0+e],c2);patch([0 0 1 1-e 0+e 0+e],[0 1 1 1-e 1-e 0+e],c3);plot([0 1 1 0 0],[0 0 1 1 0]);disp('weights');
  "IW{2,1}(80,:)'" : Constant  Value=[0.9478079839795459093920726445503532886505126953125;-0.31673347780162064424303025589324533939361572265625;-1.890888192690478586399649429949931800365447998046875;1.2749156898670095383607758776634000241756439208984375;0.09402725139458263658998049550064024515450000762939453125;-1.5645932256938752669128689376520924270153045654296875;0.07943804668258443169026605801263940520584583282470703125;-1.53590401401625431532238508225418627262115478515625]
      mask Display: e = 0.06;c1 = [120 150 230]/255;c2 = ([120 150 230]+0)/383;c3 = ([120 150 230]+128)/383;patch([0 1 1 0],[0 0 1 1],c1);patch([0 1 1 1-e 1-e 0+e],[0 0 1 1-e 0+e 0+e],c2);patch([0 0 1 1-e 0+e 0+e],[0 1 1 1-e 1-e 0+e],c3);plot([0 1 1 0 0],[0 0 1 1 0]);disp('weights');
  "IW{2,1}(800,:)'" : Constant  Value=[1.5695590533465229032827892297063954174518585205078125;1.0744248492502819214422515869955532252788543701171875;0.6560393990154651522317408307571895420551300048828125;1.74659960593104113257822973537258803844451904296875;-0.74321026821185787181178739047027193009853363037109375;-0.09591821726676737214223322780526359565556049346923828125;1.3464183066128418975182512440369464457035064697265625;1.248659653235780542246402546879835426807403564453125]
      mask Display: e = 0.06;c1 = [120 150 230]/255;c2 = ([120 150 230]+0)/383;c3 = ([120 150 230]+128)/383;patch([0 1 1 0],[0 0 1 1],c1);patch([0 1 1 1-e 1-e 0+e],[0 0 1 1-e 0+e 0+e],c2);patch([0 0 1 1-e 0+e 0+e],[0 1 1 1-e 1-e 0+e],c3);plot([0 1 1 0 0],[0 0 1 1 0]);disp('weights');
  "IW{2,1}(801,:)'" : Constant  Value=[2.0798246771491175621804359252564609050750732421875;1.4660222130354785274874984679627232253551483154296875;0.793556890082757870885643569636158645153045654296875;0.341211262274816296002910576135036535561084747314453125;0.1464014518007050458248130553329247049987316131591796875;-0.312854385738075502221278156866901554167270660400390625;-1.4814224546802143844814736439730040729045867919921875;1.21354857077294919776022652513347566127777099609375]
      mask Display: e = 0.06;c1 = [120 150 230]/255;c2 = ([120 150 230]+0)/383;c3 = ([120 150 230]+128)/383;patch([0 1 1 0],[0 0 1 1],c1);patch([0 1 1 1-e 1-e 0+e],[0 0 1 1-e 0+e 0+e],c2);patch([0 0 1 1-e 0+e 0+e],[0 1 1 1-e 1-e 0+e],c3);plot([0 1 1 0 0],[0 0 1 1 0]);disp('weights');
  "IW{2,1}(802,:)'" : Constant  Value=[-0.291074389229205976459269322731415741145610809326171875;1.9132814454774391688118839738308452069759368896484375;0.09552870719985724623501965879768249578773975372314453125;-1.8663400259594682406572019317536614835262298583984375;-1.19725755615584450453070530784316360950469970703125;0.43867878643791391457540385090396739542484283447265625;-1.38617905284088482886772908386774361133575439453125;0.519357788722857538488142381538636982440948486328125]
      mask Display: e = 0.06;c1 = [120 150 230]/255;c2 = ([120 150 230]+0)/383;c3 = ([120 150 230]+128)/383;patch([0 1 1 0],[0 0 1 1],c1);patch([0 1 1 1-e 1-e 0+e],[0 0 1 1-e 0+e 0+e],c2);patch([0 0 1 1-e 0+e 0+e],[0 1 1 1-e 1-e 0+e],c3);plot([0 1 1 0 0],[0 0 1 1 0]);disp('weights');
  "IW{2,1}(803,:)'" : Constant  Value=[1.5759999811541558489835779255372472107410430908203125;-1.33066715101493660000642194063402712345123291015625;1.0661567719787232721984082672861404716968536376953125;1.0488956736169534611491371833835728466510772705078125;0.8921151973905649956719798865378834307193756103515625;1.26977347895268533051194026484154164791107177734375;1.4620069653833793754671432907343842089176177978515625;-0.00697567377681724935800655629236644017510116100311279296875]
      mask Display: e = 0.06;c1 = [120 150 230]/255;c2 = ([120 150 230]+0)/383;c3 = ([120 150 230]+128)/383;patch([0 1 1 0],[0 0 1 1],c1);patch([0 1 1 1-e 1-e 0+e],[0 0 1 1-e 0+e 0+e],c2);patch([0 0 1 1-e 0+e 0+e],[0 1 1 1-e 1-e 0+e],c3);plot([0 1 1 0 0],[0 0 1 1 0]);disp('weights');
  "IW{2,1}(804,:)'" : Constant  Value=[-1.5331632006206203922005215645185671746730804443359375;1.616423670938370804606165620498359203338623046875;-0.269097413861498380160952592632384039461612701416015625;-1.6522077961869083839729910323512740433216094970703125;1.406510001697613976290313075878657400608062744140625;-0.5918798046138886714828686308464966714382171630859375;-0.2071267000531098745330638166706194169819355010986328125;-0.9428369908205571636727881923434324562549591064453125]
      mask Display: e = 0.06;c1 = [120 150 230]/255;c2 = ([120 150 230]+0)/383;c3 = ([120 150 230]+128)/383;patch([0 1 1 0],[0 0 1 1],c1);patch([0 1 1 1-e 1-e 0+e],[0 0 1 1-e 0+e 0+e],c2);patch([0 0 1 1-e 0+e 0+e],[0 1 1 1-e 1-e 0+e],c3);plot([0 1 1 0 0],[0 0 1 1 0]);disp('weights');
  "IW{2,1}(805,:)'" : Constant  Value=[-1.8466700241231401857788796405657194554805755615234375;-1.106214529640654919973030700930394232273101806640625;-0.58093306234666719500836506995256058871746063232421875;-0.06168916802374783958651249804461258463561534881591796875;1.5031577493678833779000569847994484007358551025390625;-0.807364994751129216865592752583324909210205078125;-1.7622619695567645070610751645290292799472808837890625;-0.15228251029610639921685333320056088268756866455078125]
      mask Display: e = 0.06;c1 = [120 150 230]/255;c2 = ([120 150 230]+0)/383;c3 = ([120 150 230]+128)/383;patch([0 1 1 0],[0 0 1 1],c1);patch([0 1 1 1-e 1-e 0+e],[0 0 1 1-e 0+e 0+e],c2);patch([0 0 1 1-e 0+e 0+e],[0 1 1 1-e 1-e 0+e],c3);plot([0 1 1 0 0],[0 0 1 1 0]);disp('weights');
  "IW{2,1}(806,:)'" : Constant  Value=[-1.47822875434379152892461206647567451000213623046875;0.72736327466593586610343891152297146618366241455078125;1.31279981257430922170215126243419945240020751953125;-1.275088111978301963489457193645648658275604248046875;-0.429694499564222731624596463007037527859210968017578125;-1.1487674103736242869899797369726002216339111328125;1.5976098856980593954091318664723075926303863525390625;0.96328808893617201558612350709154270589351654052734375]
      mask Display: e = 0.06;c1 = [120 150 230]/255;c2 = ([120 150 230]+0)/383;c3 = ([120 150 230]+128)/383;patch([0 1 1 0],[0 0 1 1],c1);patch([0 1 1 1-e 1-e 0+e],[0 0 1 1-e 0+e 0+e],c2);patch([0 0 1 1-e 0+e 0+e],[0 1 1 1-e 1-e 0+e],c3);plot([0 1 1 0 0],[0 0 1 1 0]);disp('weights');
  "IW{2,1}(807,:)'" : Constant  Value=[0.315727944716246378131785377263440750539302825927734375;0.93650927809922779321283314857282675802707672119140625;-0.77464419006669604783610338927246630191802978515625;2.129639260131461764302684969152323901653289794921875;1.698699787103432612411779700778424739837646484375;-0.1245995104072742665213269219748326577246189117431640625;-1.39309590516954973082874857936985790729522705078125;-0.283222079422675798721087403464480303227901458740234375]
      mask Display: e = 0.06;c1 = [120 150 230]/255;c2 = ([120 150 230]+0)/383;c3 = ([120 150 230]+128)/383;patch([0 1 1 0],[0 0 1 1],c1);patch([0 1 1 1-e 1-e 0+e],[0 0 1 1-e 0+e 0+e],c2);patch([0 0 1 1-e 0+e 0+e],[0 1 1 1-e 1-e 0+e],c3);plot([0 1 1 0 0],[0 0 1 1 0]);disp('weights');
  "IW{2,1}(808,:)'" : Constant  Value=[-1.5618555574041301792220792776788584887981414794921875;-1.4015706717236182665686783366254530847072601318359375;-0.9671759623680686868141265222220681607723236083984375;-1.5653136004638257272603141245781444013118743896484375;0.519447335598108406173878393019549548625946044921875;1.3042526563493572755447758027003146708011627197265625;1.032454056462201119614974231808446347713470458984375;-0.447304036868745036326089348222012631595134735107421875]
      mask Display: e = 0.06;c1 = [120 150 230]/255;c2 = ([120 150 230]+0)/383;c3 = ([120 150 230]+128)/383;patch([0 1 1 0],[0 0 1 1],c1);patch([0 1 1 1-e 1-e 0+e],[0 0 1 1-e 0+e 0+e],c2);patch([0 0 1 1-e 0+e 0+e],[0 1 1 1-e 1-e 0+e],c3);plot([0 1 1 0 0],[0 0 1 1 0]);disp('weights');
  "IW{2,1}(809,:)'" : Constant  Value=[-0.64061148040321558294607484640437178313732147216796875;0.455821452798865822675367098781862296164035797119140625;1.6715871099535071220287818505312316119670867919921875;-1.2786896327983845456088829450891353189945220947265625;-1.1969343266811931503212917959899641573429107666015625;-0.06553992843245314003919332890291116200387477874755859375;-1.63799050658778444500285331741906702518463134765625;-1.3579867239216465435447389609180390834808349609375]
      mask Display: e = 0.06;c1 = [120 150 230]/255;c2 = ([120 150 230]+0)/383;c3 = ([120 150 230]+128)/383;patch([0 1 1 0],[0 0 1 1],c1);patch([0 1 1 1-e 1-e 0+e],[0 0 1 1-e 0+e 0+e],c2);patch([0 0 1 1-e 0+e 0+e],[0 1 1 1-e 1-e 0+e],c3);plot([0 1 1 0 0],[0 0 1 1 0]);disp('weights');
  "IW{2,1}(81,:)'" : Constant  Value=[-1.26832215508676693360712306457571685314178466796875;-0.409981797206467379890426627753186039626598358154296875;-1.361928641123699268433711040415801107883453369140625;0.99313946280979947811573538274387829005718231201171875;0.426757083082677179941555323239299468696117401123046875;1.471937926405171737087584915570914745330810546875;-1.58385752210059127520480615203268826007843017578125;-1.3353107390260685605198887060396373271942138671875]
      mask Display: e = 0.06;c1 = [120 150 230]/255;c2 = ([120 150 230]+0)/383;c3 = ([120 150 230]+128)/383;patch([0 1 1 0],[0 0 1 1],c1);patch([0 1 1 1-e 1-e 0+e],[0 0 1 1-e 0+e 0+e],c2);patch([0 0 1 1-e 0+e 0+e],[0 1 1 1-e 1-e 0+e],c3);plot([0 1 1 0 0],[0 0 1 1 0]);disp('weights');
  "IW{2,1}(810,:)'" : Constant  Value=[0.87325255156883685447866128015448339283466339111328125;0.63010602895520351207636622348218224942684173583984375;1.719254592818991955738283650134690105915069580078125;0.0264765265887349186824106794801991782151162624359130859375;2.00842846918101169961801133467815816402435302734375;-0.9021620153238962824815416752244345843791961669921875;-1.2818497011301801524751908800681121647357940673828125;-0.64689828158795326107366463475045748054981231689453125]
      mask Display: e = 0.06;c1 = [120 150 230]/255;c2 = ([120 150 230]+0)/383;c3 = ([120 150 230]+128)/383;patch([0 1 1 0],[0 0 1 1],c1);patch([0 1 1 1-e 1-e 0+e],[0 0 1 1-e 0+e 0+e],c2);patch([0 0 1 1-e 0+e 0+e],[0 1 1 1-e 1-e 0+e],c3);plot([0 1 1 0 0],[0 0 1 1 0]);disp('weights');
  "IW{2,1}(811,:)'" : Constant  Value=[-1.212607417873442727795918472111225128173828125;0.23395862819571722202027785897371359169483184814453125;0.7128154408211326842348398713511414825916290283203125;1.6932202821937440972988042631186544895172119140625;-1.6052652858652027845209886436350643634796142578125;0.2535273611425676865138711946201510727405548095703125;-1.1385316436374248727503299960517324507236480712890625;-1.4761635919948254969114032064680941402912139892578125]
      mask Display: e = 0.06;c1 = [120 150 230]/255;c2 = ([120 150 230]+0)/383;c3 = ([120 150 230]+128)/383;patch([0 1 1 0],[0 0 1 1],c1);patch([0 1 1 1-e 1-e 0+e],[0 0 1 1-e 0+e 0+e],c2);patch([0 0 1 1-e 0+e 0+e],[0 1 1 1-e 1-e 0+e],c3);plot([0 1 1 0 0],[0 0 1 1 0]);disp('weights');
  "IW{2,1}(812,:)'" : Constant  Value=[0.430025388170454825331745496441726572811603546142578125;0.0229039078016529222547870148218862595967948436737060546875;-0.842140070785369676542586603318341076374053955078125;0.468236422510292460419378812730428762733936309814453125;0.362398166211760186516954718172200955450534820556640625;1.736861197339998330591015474055893719196319580078125;1.4946601591914363549307154244161210954189300537109375;2.1273209722215522532451359438709914684295654296875]
      mask Display: e = 0.06;c1 = [120 150 230]/255;c2 = ([120 150 230]+0)/383;c3 = ([120 150 230]+128)/383;patch([0 1 1 0],[0 0 1 1],c1);patch([0 1 1 1-e 1-e 0+e],[0 0 1 1-e 0+e 0+e],c2);patch([0 0 1 1-e 0+e 0+e],[0 1 1 1-e 1-e 0+e],c3);plot([0 1 1 0 0],[0 0 1 1 0]);disp('weights');
  "IW{2,1}(813,:)'" : Constant  Value=[0.115511813417477793297649668602389283478260040283203125;-1.0601456654175682725593787836260162293910980224609375;0.150624083726561941443122805139864794909954071044921875;1.098998790435593786440904295886866748332977294921875;0.234049241462977952732416042636032216250896453857421875;0.1997616802109962452771441121512907557189464569091796875;0.222254356026384158884212638440658338367938995361328125;2.91323773542059871743958865408785641193389892578125]
      mask Display: e = 0.06;c1 = [120 150 230]/255;c2 = ([120 150 230]+0)/383;c3 = ([120 150 230]+128)/383;patch([0 1 1 0],[0 0 1 1],c1);patch([0 1 1 1-e 1-e 0+e],[0 0 1 1-e 0+e 0+e],c2);patch([0 0 1 1-e 0+e 0+e],[0 1 1 1-e 1-e 0+e],c3);plot([0 1 1 0 0],[0 0 1 1 0]);disp('weights');
  "IW{2,1}(814,:)'" : Constant  Value=[0.044624415338747801251795266352928592823445796966552734375;-0.52758196424207592922783760513993911445140838623046875;1.7771384278490101049641225472441874444484710693359375;-1.9220048346653031412500922670005820691585540771484375;0.339500999097111844093888066709041595458984375;-1.25734577675718472988819485181011259555816650390625;1.34201829296861152585051968344487249851226806640625;-0.4651445739697523951150515131303109228610992431640625]
      mask Display: e = 0.06;c1 = [120 150 230]/255;c2 = ([120 150 230]+0)/383;c3 = ([120 150 230]+128)/383;patch([0 1 1 0],[0 0 1 1],c1);patch([0 1 1 1-e 1-e 0+e],[0 0 1 1-e 0+e 0+e],c2);patch([0 0 1 1-e 0+e 0+e],[0 1 1 1-e 1-e 0+e],c3);plot([0 1 1 0 0],[0 0 1 1 0]);disp('weights');
  "IW{2,1}(815,:)'" : Constant  Value=[-1.5480154775468306649344185643712989985942840576171875;1.034048195283008286793346997001208364963531494140625;-0.7247839706364416212380774595658294856548309326171875;-1.2943573348302963577083346535800956189632415771484375;-1.385788860170300562657530463184230029582977294921875;1.1098507096010779005013091591536067426204681396484375;-1.0821042645753495836657975814887322485446929931640625;1.0137282500325230927273878478445112705230712890625]
      mask Display: e = 0.06;c1 = [120 150 230]/255;c2 = ([120 150 230]+0)/383;c3 = ([120 150 230]+128)/383;patch([0 1 1 0],[0 0 1 1],c1);patch([0 1 1 1-e 1-e 0+e],[0 0 1 1-e 0+e 0+e],c2);patch([0 0 1 1-e 0+e 0+e],[0 1 1 1-e 1-e 0+e],c3);plot([0 1 1 0 0],[0 0 1 1 0]);disp('weights');
  "IW{2,1}(816,:)'" : Constant  Value=[-1.7508619714869073646923425258137285709381103515625;-1.586820481976472851926018847734667360782623291015625;-0.1941993105663601948407404051977209746837615966796875;-0.74026805770250991844960708476719446480274200439453125;0.556144062760079993523731900495477020740509033203125;1.76289438682278909453771120752207934856414794921875;-0.377691270619008701014962525732698850333690643310546875;-1.133625897620685218925018489244394004344940185546875]
      mask Display: e = 0.06;c1 = [120 150 230]/255;c2 = ([120 150 230]+0)/383;c3 = ([120 150 230]+128)/383;patch([0 1 1 0],[0 0 1 1],c1);patch([0 1 1 1-e 1-e 0+e],[0 0 1 1-e 0+e 0+e],c2);patch([0 0 1 1-e 0+e 0+e],[0 1 1 1-e 1-e 0+e],c3);plot([0 1 1 0 0],[0 0 1 1 0]);disp('weights');
  "IW{2,1}(817,:)'" : Constant  Value=[0.5343707506379373750604599990765564143657684326171875;-0.75947253303242201472045280752354301512241363525390625;-1.69087515744136585027490582433529198169708251953125;1.609678994617831815361341796233318746089935302734375;-1.000180913614647781884059440926648676395416259765625;-1.911273437576257894221498645492829382419586181640625;0.04239258308060013524798392836601124145090579986572265625;-0.362515329955529763683585997569025494158267974853515625]
      mask Display: e = 0.06;c1 = [120 150 230]/255;c2 = ([120 150 230]+0)/383;c3 = ([120 150 230]+128)/383;patch([0 1 1 0],[0 0 1 1],c1);patch([0 1 1 1-e 1-e 0+e],[0 0 1 1-e 0+e 0+e],c2);patch([0 0 1 1-e 0+e 0+e],[0 1 1 1-e 1-e 0+e],c3);plot([0 1 1 0 0],[0 0 1 1 0]);disp('weights');
  "IW{2,1}(818,:)'" : Constant  Value=[0.7283650437795843313182331257849000394344329833984375;-1.9961665022618575449087074957787990570068359375;0.364472854566094628392391996385413222014904022216796875;1.120015199326426458270589137100614607334136962890625;0.59917264989503393746161918897996656596660614013671875;1.027905959856982409661441124626435339450836181640625;0.51278702111671725649699737914488650858402252197265625;1.856056038754456238848433713428676128387451171875]
      mask Display: e = 0.06;c1 = [120 150 230]/255;c2 = ([120 150 230]+0)/383;c3 = ([120 150 230]+128)/383;patch([0 1 1 0],[0 0 1 1],c1);patch([0 1 1 1-e 1-e 0+e],[0 0 1 1-e 0+e 0+e],c2);patch([0 0 1 1-e 0+e 0+e],[0 1 1 1-e 1-e 0+e],c3);plot([0 1 1 0 0],[0 0 1 1 0]);disp('weights');
  "IW{2,1}(819,:)'" : Constant  Value=[1.1456779075445850946124437541584484279155731201171875;0.88212488716016312917389541325974278151988983154296875;0.36487779083907601052061409063753671944141387939453125;-1.22404070840442091849809003178961575031280517578125;-0.76113816291248193035556823815568350255489349365234375;0.83545174209844208501607454309123568236827850341796875;1.682168954731877885677704398403875529766082763671875;-1.7773792648860424758794351873802952468395233154296875]
      mask Display: e = 0.06;c1 = [120 150 230]/255;c2 = ([120 150 230]+0)/383;c3 = ([120 150 230]+128)/383;patch([0 1 1 0],[0 0 1 1],c1);patch([0 1 1 1-e 1-e 0+e],[0 0 1 1-e 0+e 0+e],c2);patch([0 0 1 1-e 0+e 0+e],[0 1 1 1-e 1-e 0+e],c3);plot([0 1 1 0 0],[0 0 1 1 0]);disp('weights');
  "IW{2,1}(82,:)'" : Constant  Value=[2.101329974583277415689508416107855737209320068359375;-1.124226133762953327988043383811600506305694580078125;-0.1414973703938578186711794160146382637321949005126953125;-1.2816701396759755393617297158925794064998626708984375;1.1702270670809580277449413188151083886623382568359375;1.1664148835574768003908729951945133507251739501953125;-0.7900983659970943762118622544221580028533935546875;0.74416803272525011703208974722656421363353729248046875]
      mask Display: e = 0.06;c1 = [120 150 230]/255;c2 = ([120 150 230]+0)/383;c3 = ([120 150 230]+128)/383;patch([0 1 1 0],[0 0 1 1],c1);patch([0 1 1 1-e 1-e 0+e],[0 0 1 1-e 0+e 0+e],c2);patch([0 0 1 1-e 0+e 0+e],[0 1 1 1-e 1-e 0+e],c3);plot([0 1 1 0 0],[0 0 1 1 0]);disp('weights');
  "IW{2,1}(820,:)'" : Constant  Value=[-1.500489075953748141500909696333110332489013671875;0.7206186522256856630264110208372585475444793701171875;-1.167302690367808093441226446884684264659881591796875;0.93036001603113482882889684333349578082561492919921875;-1.34005957253632601577919558621942996978759765625;-1.097093076011818713055845364578999578952789306640625;-1.680600487692627265090550281456671655178070068359375;0.43978169098418529170402280215057544410228729248046875]
      mask Display: e = 0.06;c1 = [120 150 230]/255;c2 = ([120 150 230]+0)/383;c3 = ([120 150 230]+128)/383;patch([0 1 1 0],[0 0 1 1],c1);patch([0 1 1 1-e 1-e 0+e],[0 0 1 1-e 0+e 0+e],c2);patch([0 0 1 1-e 0+e 0+e],[0 1 1 1-e 1-e 0+e],c3);plot([0 1 1 0 0],[0 0 1 1 0]);disp('weights');
  "IW{2,1}(821,:)'" : Constant  Value=[-0.66422170217768705668959228205494582653045654296875;0.0396151629278536365763585536114987917244434356689453125;1.4553922222335333724885231276857666671276092529296875;0.261012957706985293526713576284237205982208251953125;1.37657210719146139155100172501988708972930908203125;2.462232963326156376382414237014017999172210693359375;0.710605878783713951207801073906011879444122314453125;0.01490518553212233192339919440883022616617381572723388671875]
      mask Display: e = 0.06;c1 = [120 150 230]/255;c2 = ([120 150 230]+0)/383;c3 = ([120 150 230]+128)/383;patch([0 1 1 0],[0 0 1 1],c1);patch([0 1 1 1-e 1-e 0+e],[0 0 1 1-e 0+e 0+e],c2);patch([0 0 1 1-e 0+e 0+e],[0 1 1 1-e 1-e 0+e],c3);plot([0 1 1 0 0],[0 0 1 1 0]);disp('weights');
  "IW{2,1}(822,:)'" : Constant  Value=[-0.83157377001387888793004776744055561721324920654296875;0.7435851961764934348053657231503166258335113525390625;-1.82463925339214227960837888531386852264404296875;-1.7317470141051998222536667526583187282085418701171875;0.400068023166359865161467723737587220966815948486328125;-0.99267113546551455360855698017985559999942779541015625;0.9593520084312727735920134364278055727481842041015625;-1.175456095935742961700043451855890452861785888671875]
      mask Display: e = 0.06;c1 = [120 150 230]/255;c2 = ([120 150 230]+0)/383;c3 = ([120 150 230]+128)/383;patch([0 1 1 0],[0 0 1 1],c1);patch([0 1 1 1-e 1-e 0+e],[0 0 1 1-e 0+e 0+e],c2);patch([0 0 1 1-e 0+e 0+e],[0 1 1 1-e 1-e 0+e],c3);plot([0 1 1 0 0],[0 0 1 1 0]);disp('weights');
  "IW{2,1}(823,:)'" : Constant  Value=[-0.265474726171173236455302912872866727411746978759765625;-2.0885097264814529438581303111277520656585693359375;-0.06488111573959109978915194005821831524372100830078125;0.294663815795885575266055411702836863696575164794921875;-1.4505703516766763616629987154738046228885650634765625;0.96833042647942024760965296081849373877048492431640625;1.1133809027849839168311518733389675617218017578125;1.4823027023776234045726596377789974212646484375]
      mask Display: e = 0.06;c1 = [120 150 230]/255;c2 = ([120 150 230]+0)/383;c3 = ([120 150 230]+128)/383;patch([0 1 1 0],[0 0 1 1],c1);patch([0 1 1 1-e 1-e 0+e],[0 0 1 1-e 0+e 0+e],c2);patch([0 0 1 1-e 0+e 0+e],[0 1 1 1-e 1-e 0+e],c3);plot([0 1 1 0 0],[0 0 1 1 0]);disp('weights');
  "IW{2,1}(824,:)'" : Constant  Value=[-0.5658108615650963013621321806567721068859100341796875;1.5917202526154639041777727470616810023784637451171875;-1.061790306112855741815792498528026044368743896484375;-0.7207746794024936232148093040450476109981536865234375;-0.97659918811447166131500807750853709876537322998046875;1.537999849976440014387435439857654273509979248046875;1.6851516824111616443815364618785679340362548828125;0.3167726592597002177598142225178889930248260498046875]
      mask Display: e = 0.06;c1 = [120 150 230]/255;c2 = ([120 150 230]+0)/383;c3 = ([120 150 230]+128)/383;patch([0 1 1 0],[0 0 1 1],c1);patch([0 1 1 1-e 1-e 0+e],[0 0 1 1-e 0+e 0+e],c2);patch([0 0 1 1-e 0+e 0+e],[0 1 1 1-e 1-e 0+e],c3);plot([0 1 1 0 0],[0 0 1 1 0]);disp('weights');
  "IW{2,1}(825,:)'" : Constant  Value=[-0.1748236010427055286964304059438291005790233612060546875;-1.4223722138761303313003736548125743865966796875;-0.69800158547010260345899723688489757478237152099609375;-2.16935583369800877306943220901302993297576904296875;1.68126589143772520174024975858628749847412109375;0.144983449537851860622339472683961503207683563232421875;-0.89463807068714495951411436180933378636837005615234375;0.33298654819377115909873054988565854728221893310546875]
      mask Display: e = 0.06;c1 = [120 150 230]/255;c2 = ([120 150 230]+0)/383;c3 = ([120 150 230]+128)/383;patch([0 1 1 0],[0 0 1 1],c1);patch([0 1 1 1-e 1-e 0+e],[0 0 1 1-e 0+e 0+e],c2);patch([0 0 1 1-e 0+e 0+e],[0 1 1 1-e 1-e 0+e],c3);plot([0 1 1 0 0],[0 0 1 1 0]);disp('weights');
  "IW{2,1}(826,:)'" : Constant  Value=[0.853239127151329768139476072974503040313720703125;0.59188819040715212604908401772263459861278533935546875;-2.157649064705599695201954091317020356655120849609375;1.0548156189125332815592628321610391139984130859375;-1.8589092283988331022470674724900163710117340087890625;-0.363367657711652913832267586258240044116973876953125;0.420258921554142406140641696765669621527194976806640625;-0.68222416774334837530346931089297868311405181884765625]
      mask Display: e = 0.06;c1 = [120 150 230]/255;c2 = ([120 150 230]+0)/383;c3 = ([120 150 230]+128)/383;patch([0 1 1 0],[0 0 1 1],c1);patch([0 1 1 1-e 1-e 0+e],[0 0 1 1-e 0+e 0+e],c2);patch([0 0 1 1-e 0+e 0+e],[0 1 1 1-e 1-e 0+e],c3);plot([0 1 1 0 0],[0 0 1 1 0]);disp('weights');
  "IW{2,1}(827,:)'" : Constant  Value=[-0.0439241990813858673714520364228519611060619354248046875;-0.4913856620836909439020701029221527278423309326171875;1.5402925110626968230320699149160645902156829833984375;1.620107617907802666223915366572327911853790283203125;-1.3250874645916013161439650502870790660381317138671875;-1.9999435258619178146233252846286632120609283447265625;-0.385254484933126140067116693899151869118213653564453125;0.0425462599664178375835632550661102868616580963134765625]
      mask Display: e = 0.06;c1 = [120 150 230]/255;c2 = ([120 150 230]+0)/383;c3 = ([120 150 230]+128)/383;patch([0 1 1 0],[0 0 1 1],c1);patch([0 1 1 1-e 1-e 0+e],[0 0 1 1-e 0+e 0+e],c2);patch([0 0 1 1-e 0+e 0+e],[0 1 1 1-e 1-e 0+e],c3);plot([0 1 1 0 0],[0 0 1 1 0]);disp('weights');
  "IW{2,1}(828,:)'" : Constant  Value=[-1.8172313004963240867795093436143361032009124755859375;1.7455399824441908407379742129705846309661865234375;0.2745373028465312170709466954576782882213592529296875;0.00013359351510363619741812712948814123592455871403217315673828125;-1.8798769733719280505823689964017830789089202880859375;-0.77255312045982116320175236978684552013874053955078125;-0.27064835130874065338701939253951422870159149169921875;-0.61166173152475489249724205365055240690708160400390625]
      mask Display: e = 0.06;c1 = [120 150 230]/255;c2 = ([120 150 230]+0)/383;c3 = ([120 150 230]+128)/383;patch([0 1 1 0],[0 0 1 1],c1);patch([0 1 1 1-e 1-e 0+e],[0 0 1 1-e 0+e 0+e],c2);patch([0 0 1 1-e 0+e 0+e],[0 1 1 1-e 1-e 0+e],c3);plot([0 1 1 0 0],[0 0 1 1 0]);disp('weights');
  "IW{2,1}(829,:)'" : Constant  Value=[-1.650212628942254067254680194309912621974945068359375;1.54724486977550679256410148809663951396942138671875;-1.6687925542211592411234732935554347932338714599609375;-0.903506718287258703270481419167481362819671630859375;-0.50860824732043941054371316567994654178619384765625;-0.68368206350197535670076831593178212642669677734375;1.226984393512414062143989212927408516407012939453125;-0.06276246456883551039229729440194205380976200103759765625]
      mask Display: e = 0.06;c1 = [120 150 230]/255;c2 = ([120 150 230]+0)/383;c3 = ([120 150 230]+128)/383;patch([0 1 1 0],[0 0 1 1],c1);patch([0 1 1 1-e 1-e 0+e],[0 0 1 1-e 0+e 0+e],c2);patch([0 0 1 1-e 0+e 0+e],[0 1 1 1-e 1-e 0+e],c3);plot([0 1 1 0 0],[0 0 1 1 0]);disp('weights');
  "IW{2,1}(83,:)'" : Constant  Value=[0.431363094706028127323094167877570725977420806884765625;1.9265269950132604126480373452068306505680084228515625;-0.7579094692078347517139036426669918000698089599609375;0.4865127646217459744804045840282924473285675048828125;-0.26598145627575553451293899342999793589115142822265625;1.3763325032036137773872042089351452887058258056640625;-1.1944355271512374638831488482537679374217987060546875;-1.6995858486232189310527473935508169233798980712890625]
      mask Display: e = 0.06;c1 = [120 150 230]/255;c2 = ([120 150 230]+0)/383;c3 = ([120 150 230]+128)/383;patch([0 1 1 0],[0 0 1 1],c1);patch([0 1 1 1-e 1-e 0+e],[0 0 1 1-e 0+e 0+e],c2);patch([0 0 1 1-e 0+e 0+e],[0 1 1 1-e 1-e 0+e],c3);plot([0 1 1 0 0],[0 0 1 1 0]);disp('weights');
  "IW{2,1}(830,:)'" : Constant  Value=[0.86618119244503011255886804065085016191005706787109375;-1.063791004447411925326605341979302465915679931640625;0.28071579925086276308121568945352919399738311767578125;-0.55894803333170595127654678435646928846836090087890625;1.3520999247321372482844026308157481253147125244140625;-0.3023806288223911398205245859571732580661773681640625;1.800170322078616269578787978389300405979156494140625;-1.902760363030104873161008072202093899250030517578125]
      mask Display: e = 0.06;c1 = [120 150 230]/255;c2 = ([120 150 230]+0)/383;c3 = ([120 150 230]+128)/383;patch([0 1 1 0],[0 0 1 1],c1);patch([0 1 1 1-e 1-e 0+e],[0 0 1 1-e 0+e 0+e],c2);patch([0 0 1 1-e 0+e 0+e],[0 1 1 1-e 1-e 0+e],c3);plot([0 1 1 0 0],[0 0 1 1 0]);disp('weights');
  "IW{2,1}(831,:)'" : Constant  Value=[-0.59612265693842714231465151897282339632511138916015625;0.5474328439348408181785998749546706676483154296875;-0.299743600840427226739137722688610665500164031982421875;1.6739951687401226632090356361004523932933807373046875;0.8045159342709287120243288882193155586719512939453125;1.9441548402720207899818660735036246478557586669921875;1.0122169128063502885339630665839649736881256103515625;-1.44063032901432652721496197045780718326568603515625]
      mask Display: e = 0.06;c1 = [120 150 230]/255;c2 = ([120 150 230]+0)/383;c3 = ([120 150 230]+128)/383;patch([0 1 1 0],[0 0 1 1],c1);patch([0 1 1 1-e 1-e 0+e],[0 0 1 1-e 0+e 0+e],c2);patch([0 0 1 1-e 0+e 0+e],[0 1 1 1-e 1-e 0+e],c3);plot([0 1 1 0 0],[0 0 1 1 0]);disp('weights');
  "IW{2,1}(832,:)'" : Constant  Value=[-1.4762470812068404502070961825666017830371856689453125;-0.441887055750879997884084104953217320144176483154296875;-0.369931344033229747569890832892269827425479888916015625;-1.0533545749347326125899826365639455616474151611328125;1.3969128720635008988892877823673188686370849609375;-1.324852004396026128318908376968465745449066162109375;1.5038442231756936617870223926729522645473480224609375;1.160829550127791431890500462031923234462738037109375]
      mask Display: e = 0.06;c1 = [120 150 230]/255;c2 = ([120 150 230]+0)/383;c3 = ([120 150 230]+128)/383;patch([0 1 1 0],[0 0 1 1],c1);patch([0 1 1 1-e 1-e 0+e],[0 0 1 1-e 0+e 0+e],c2);patch([0 0 1 1-e 0+e 0+e],[0 1 1 1-e 1-e 0+e],c3);plot([0 1 1 0 0],[0 0 1 1 0]);disp('weights');
  "IW{2,1}(833,:)'" : Constant  Value=[-1.5041988287399792323384417613851837813854217529296875;1.544194754049979412258153388393111526966094970703125;2.04764594963646562320036537130363285541534423828125;0.006256524374803863579319607168827133136801421642303466796875;1.0017559886360789533910065074451267719268798828125;0.223271184523280652456378447823226451873779296875;0.71744096989837391475930417072959244251251220703125;-0.6553627804670594247937742693466134369373321533203125]
      mask Display: e = 0.06;c1 = [120 150 230]/255;c2 = ([120 150 230]+0)/383;c3 = ([120 150 230]+128)/383;patch([0 1 1 0],[0 0 1 1],c1);patch([0 1 1 1-e 1-e 0+e],[0 0 1 1-e 0+e 0+e],c2);patch([0 0 1 1-e 0+e 0+e],[0 1 1 1-e 1-e 0+e],c3);plot([0 1 1 0 0],[0 0 1 1 0]);disp('weights');
  "IW{2,1}(834,:)'" : Constant  Value=[-1.7354828331888663139892514664097689092159271240234375;-0.0190194373071912968542473976185647188685834407806396484375;0.295580091036368564072489562022383324801921844482421875;-0.27339801390655082968805800192058086395263671875;-1.553139641288189043422107715741731226444244384765625;-0.9211946162753685829471805845969356596469879150390625;2.040431418905929827900536110973916947841644287109375;-0.6534862581096103628652826955658383667469024658203125]
      mask Display: e = 0.06;c1 = [120 150 230]/255;c2 = ([120 150 230]+0)/383;c3 = ([120 150 230]+128)/383;patch([0 1 1 0],[0 0 1 1],c1);patch([0 1 1 1-e 1-e 0+e],[0 0 1 1-e 0+e 0+e],c2);patch([0 0 1 1-e 0+e 0+e],[0 1 1 1-e 1-e 0+e],c3);plot([0 1 1 0 0],[0 0 1 1 0]);disp('weights');
  "IW{2,1}(835,:)'" : Constant  Value=[-1.4267357384755967597556036707828752696514129638671875;-1.4990752442383741271925146065768785774707794189453125;-0.5218991518188025313662592452601529657840728759765625;1.7379049954773104769145675163599662482738494873046875;-0.2123833265105544987338959117550984956324100494384765625;0.77087333807097924154305701449629850685596466064453125;1.4403274972092894312680755319888703525066375732421875;-0.89369907698194406275860046662273816764354705810546875]
      mask Display: e = 0.06;c1 = [120 150 230]/255;c2 = ([120 150 230]+0)/383;c3 = ([120 150 230]+128)/383;patch([0 1 1 0],[0 0 1 1],c1);patch([0 1 1 1-e 1-e 0+e],[0 0 1 1-e 0+e 0+e],c2);patch([0 0 1 1-e 0+e 0+e],[0 1 1 1-e 1-e 0+e],c3);plot([0 1 1 0 0],[0 0 1 1 0]);disp('weights');
  "IW{2,1}(836,:)'" : Constant  Value=[-0.99554450876987043983490366372279822826385498046875;-1.6788898987260323369952175198704935610294342041015625;-0.202720926791548572420964546836330555379390716552734375;-0.855022448048981420498648731154389679431915283203125;-1.8826335935391707021580032233032397925853729248046875;-1.473845768980613701870652221259661018848419189453125;0.280231849864717441622730120798223651945590972900390625;0.80031895304259415002690047913347370922565460205078125]
      mask Display: e = 0.06;c1 = [120 150 230]/255;c2 = ([120 150 230]+0)/383;c3 = ([120 150 230]+128)/383;patch([0 1 1 0],[0 0 1 1],c1);patch([0 1 1 1-e 1-e 0+e],[0 0 1 1-e 0+e 0+e],c2);patch([0 0 1 1-e 0+e 0+e],[0 1 1 1-e 1-e 0+e],c3);plot([0 1 1 0 0],[0 0 1 1 0]);disp('weights');
  "IW{2,1}(837,:)'" : Constant  Value=[0.06798555638648069721075017923794803209602832794189453125;-1.64161938848386501632603540201671421527862548828125;1.88201844569940757168069467297755181789398193359375;-0.1066197818126391749782300166771165095269680023193359375;-1.0446015686215457396457395589095540344715118408203125;-0.06404654682422615541437238562139100395143032073974609375;1.0472690184596913365311365851084701716899871826171875;1.6003431666075156325490524977794848382472991943359375]
      mask Display: e = 0.06;c1 = [120 150 230]/255;c2 = ([120 150 230]+0)/383;c3 = ([120 150 230]+128)/383;patch([0 1 1 0],[0 0 1 1],c1);patch([0 1 1 1-e 1-e 0+e],[0 0 1 1-e 0+e 0+e],c2);patch([0 0 1 1-e 0+e 0+e],[0 1 1 1-e 1-e 0+e],c3);plot([0 1 1 0 0],[0 0 1 1 0]);disp('weights');
  "IW{2,1}(838,:)'" : Constant  Value=[-0.41624932511491241626799819641746580600738525390625;0.04576611604644058306501364086216199211776256561279296875;1.8372331869610476484666605756501667201519012451171875;0.81992081079686585098897921852767467498779296875;-1.795986524679220597278117566020227968692779541015625;-0.8600294213468633319763512190547771751880645751953125;-0.8562435616058514664672429717029444873332977294921875;-1.453141521768305022277445459621958434581756591796875]
      mask Display: e = 0.06;c1 = [120 150 230]/255;c2 = ([120 150 230]+0)/383;c3 = ([120 150 230]+128)/383;patch([0 1 1 0],[0 0 1 1],c1);patch([0 1 1 1-e 1-e 0+e],[0 0 1 1-e 0+e 0+e],c2);patch([0 0 1 1-e 0+e 0+e],[0 1 1 1-e 1-e 0+e],c3);plot([0 1 1 0 0],[0 0 1 1 0]);disp('weights');
  "IW{2,1}(839,:)'" : Constant  Value=[0.6769471956063226603106386392028070986270904541015625;-1.65300496471176305846029208623804152011871337890625;-1.42115956800614551269745788886211812496185302734375;-1.480277131739204943272625314421020448207855224609375;-1.0043142204916410964443684861180372536182403564453125;0.06463614344972068437300549703650176525115966796875;1.2374550227295568749497078897547908127307891845703125;-0.90192689639029610670917236348032020032405853271484375]
      mask Display: e = 0.06;c1 = [120 150 230]/255;c2 = ([120 150 230]+0)/383;c3 = ([120 150 230]+128)/383;patch([0 1 1 0],[0 0 1 1],c1);patch([0 1 1 1-e 1-e 0+e],[0 0 1 1-e 0+e 0+e],c2);patch([0 0 1 1-e 0+e 0+e],[0 1 1 1-e 1-e 0+e],c3);plot([0 1 1 0 0],[0 0 1 1 0]);disp('weights');
  "IW{2,1}(84,:)'" : Constant  Value=[0.8992620690505914726742275888682343065738677978515625;-0.018726788154049330004102813518329639919102191925048828125;-1.3766172853565123990193796998937614262104034423828125;0.8878833742337042256309587173745967447757720947265625;-1.6388784375125495795799679399351589381694793701171875;-0.51337464096851181949432429973967373371124267578125;1.632592883272429684637927493895404040813446044921875;-1.3899514300105282327280065146624110639095306396484375]
      mask Display: e = 0.06;c1 = [120 150 230]/255;c2 = ([120 150 230]+0)/383;c3 = ([120 150 230]+128)/383;patch([0 1 1 0],[0 0 1 1],c1);patch([0 1 1 1-e 1-e 0+e],[0 0 1 1-e 0+e 0+e],c2);patch([0 0 1 1-e 0+e 0+e],[0 1 1 1-e 1-e 0+e],c3);plot([0 1 1 0 0],[0 0 1 1 0]);disp('weights');
  "IW{2,1}(840,:)'" : Constant  Value=[1.773732461014815076083550593466497957706451416015625;0.7529353002482699341868510600761510431766510009765625;0.6541016959312988543473466052091680467128753662109375;0.8184720081703875660394942315178923308849334716796875;1.1222689000190204655638126496342010796070098876953125;-1.0279935713869685631749462118023075163364410400390625;1.91052916390469729179812929942272603511810302734375;0.495408483372323737992104497607215307652950286865234375]
      mask Display: e = 0.06;c1 = [120 150 230]/255;c2 = ([120 150 230]+0)/383;c3 = ([120 150 230]+128)/383;patch([0 1 1 0],[0 0 1 1],c1);patch([0 1 1 1-e 1-e 0+e],[0 0 1 1-e 0+e 0+e],c2);patch([0 0 1 1-e 0+e 0+e],[0 1 1 1-e 1-e 0+e],c3);plot([0 1 1 0 0],[0 0 1 1 0]);disp('weights');
  "IW{2,1}(841,:)'" : Constant  Value=[0.24436535503291756388222211171523667871952056884765625;-1.137442492085455558736839520861394703388214111328125;-1.2741845569837073615104827695176936686038970947265625;1.84744514399857440167806998942978680133819580078125;1.3756451076393869659142410455388016998767852783203125;-0.360834248794258793946454488832387141883373260498046875;0.04735775656772837904906481298894505016505718231201171875;-1.560049966069621429909375365241430699825286865234375]
      mask Display: e = 0.06;c1 = [120 150 230]/255;c2 = ([120 150 230]+0)/383;c3 = ([120 150 230]+128)/383;patch([0 1 1 0],[0 0 1 1],c1);patch([0 1 1 1-e 1-e 0+e],[0 0 1 1-e 0+e 0+e],c2);patch([0 0 1 1-e 0+e 0+e],[0 1 1 1-e 1-e 0+e],c3);plot([0 1 1 0 0],[0 0 1 1 0]);disp('weights');
  "IW{2,1}(842,:)'" : Constant  Value=[-0.6493631114617557376078593733836896717548370361328125;1.808643656557480827729023076244629919528961181640625;-1.1265193434280906803479638256249018013477325439453125;0.9486822290369871790716160830925218760967254638671875;0.50069194363258306967878752402612008154392242431640625;1.940636625400891990267382425372488796710968017578125;0.5191715207024236722332943827495910227298736572265625;1.0221937408713159811668447218835353851318359375]
      mask Display: e = 0.06;c1 = [120 150 230]/255;c2 = ([120 150 230]+0)/383;c3 = ([120 150 230]+128)/383;patch([0 1 1 0],[0 0 1 1],c1);patch([0 1 1 1-e 1-e 0+e],[0 0 1 1-e 0+e 0+e],c2);patch([0 0 1 1-e 0+e 0+e],[0 1 1 1-e 1-e 0+e],c3);plot([0 1 1 0 0],[0 0 1 1 0]);disp('weights');
  "IW{2,1}(843,:)'" : Constant  Value=[1.1132295610347515690818909206427633762359619140625;1.265008390658156400832012877799570560455322265625;-1.7841447835237875807479213108308613300323486328125;1.106941978420424188556125955074094235897064208984375;0.76261572839963054359913030566531233489513397216796875;-1.0729668090216490927701897817314602434635162353515625;0.6274850309355459732074677958735264837741851806640625;1.285491774131467312969334670924581587314605712890625]
      mask Display: e = 0.06;c1 = [120 150 230]/255;c2 = ([120 150 230]+0)/383;c3 = ([120 150 230]+128)/383;patch([0 1 1 0],[0 0 1 1],c1);patch([0 1 1 1-e 1-e 0+e],[0 0 1 1-e 0+e 0+e],c2);patch([0 0 1 1-e 0+e 0+e],[0 1 1 1-e 1-e 0+e],c3);plot([0 1 1 0 0],[0 0 1 1 0]);disp('weights');
  "IW{2,1}(844,:)'" : Constant  Value=[1.1202035089892614649897950585000216960906982421875;-0.63887774059653279490333943613222800195217132568359375;0.6432878091338860571113400510512292385101318359375;1.6760332357238432177126696842606179416179656982421875;-0.148940673252003608073579243864514864981174468994140625;1.543624662575144412812733207829296588897705078125;-1.854071925955321997747660134336911141872406005859375;-0.54983090107711796168388218575273640453815460205078125]
      mask Display: e = 0.06;c1 = [120 150 230]/255;c2 = ([120 150 230]+0)/383;c3 = ([120 150 230]+128)/383;patch([0 1 1 0],[0 0 1 1],c1);patch([0 1 1 1-e 1-e 0+e],[0 0 1 1-e 0+e 0+e],c2);patch([0 0 1 1-e 0+e 0+e],[0 1 1 1-e 1-e 0+e],c3);plot([0 1 1 0 0],[0 0 1 1 0]);disp('weights');
  "IW{2,1}(845,:)'" : Constant  Value=[0.016301555419528275525653526756286737509071826934814453125;-0.8553777683528844821836401024484075605869293212890625;1.5785643831236111367388730286620557308197021484375;1.84359947055318595943163018091581761837005615234375;-0.1851666373078672267471489476520218886435031890869140625;1.878186362007655763051161557086743414402008056640625;-0.10226129310859662091548472062640939839184284210205078125;0.9142805504110651515503604969126172363758087158203125]
      mask Display: e = 0.06;c1 = [120 150 230]/255;c2 = ([120 150 230]+0)/383;c3 = ([120 150 230]+128)/383;patch([0 1 1 0],[0 0 1 1],c1);patch([0 1 1 1-e 1-e 0+e],[0 0 1 1-e 0+e 0+e],c2);patch([0 0 1 1-e 0+e 0+e],[0 1 1 1-e 1-e 0+e],c3);plot([0 1 1 0 0],[0 0 1 1 0]);disp('weights');
  "IW{2,1}(846,:)'" : Constant  Value=[-0.262061438918995748270646117816795594990253448486328125;1.0911657301071746584142374558723531663417816162109375;-0.6790408173144282244493297184817492961883544921875;-2.101417211277741170505350964958779513835906982421875;2.088108555647333997029591046157293021678924560546875;0.097517306804930481423099308813107199966907501220703125;-0.85575185233957729025178196025080978870391845703125;-0.033384931598316132383974519370894995518028736114501953125]
      mask Display: e = 0.06;c1 = [120 150 230]/255;c2 = ([120 150 230]+0)/383;c3 = ([120 150 230]+128)/383;patch([0 1 1 0],[0 0 1 1],c1);patch([0 1 1 1-e 1-e 0+e],[0 0 1 1-e 0+e 0+e],c2);patch([0 0 1 1-e 0+e 0+e],[0 1 1 1-e 1-e 0+e],c3);plot([0 1 1 0 0],[0 0 1 1 0]);disp('weights');
  "IW{2,1}(847,:)'" : Constant  Value=[0.155721308226543342367875766285578720271587371826171875;-0.8846703173677850084999363389215432107448577880859375;0.56178200623051333106872107236995361745357513427734375;1.30867862300235504591228163917548954486846923828125;-1.704606717393348791489415816613472998142242431640625;-1.0642321493165145529502524368581362068653106689453125;1.8064452206998371508461787016130983829498291015625;1.000006437500949640906355853076092898845672607421875]
      mask Display: e = 0.06;c1 = [120 150 230]/255;c2 = ([120 150 230]+0)/383;c3 = ([120 150 230]+128)/383;patch([0 1 1 0],[0 0 1 1],c1);patch([0 1 1 1-e 1-e 0+e],[0 0 1 1-e 0+e 0+e],c2);patch([0 0 1 1-e 0+e 0+e],[0 1 1 1-e 1-e 0+e],c3);plot([0 1 1 0 0],[0 0 1 1 0]);disp('weights');
  "IW{2,1}(848,:)'" : Constant  Value=[0.1650307156086321669352656726914574392139911651611328125;2.035696567717259153340592092717997729778289794921875;-1.173871216712292220307745083118788897991180419921875;0.0231494191358121124968416637557311332784593105316162109375;0.76960602845755865519805638541583903133869171142578125;-1.3854331403439292813573047169484198093414306640625;-1.040709879775010282543235007324256002902984619140625;-1.3180058969331669427305087083368562161922454833984375]
      mask Display: e = 0.06;c1 = [120 150 230]/255;c2 = ([120 150 230]+0)/383;c3 = ([120 150 230]+128)/383;patch([0 1 1 0],[0 0 1 1],c1);patch([0 1 1 1-e 1-e 0+e],[0 0 1 1-e 0+e 0+e],c2);patch([0 0 1 1-e 0+e 0+e],[0 1 1 1-e 1-e 0+e],c3);plot([0 1 1 0 0],[0 0 1 1 0]);disp('weights');
  "IW{2,1}(849,:)'" : Constant  Value=[0.62780727117172097084818460643873549997806549072265625;1.5121040852257887632248412046465091407299041748046875;1.53432921839906644123630030662752687931060791015625;-1.8220253389407192745608199402340687811374664306640625;0.64801890338045586847925960682914592325687408447265625;1.2644775992963419586345708012231625616550445556640625;0.1399288111750844609826316400358336977660655975341796875;-0.806956304519284461918005035840906202793121337890625]
      mask Display: e = 0.06;c1 = [120 150 230]/255;c2 = ([120 150 230]+0)/383;c3 = ([120 150 230]+128)/383;patch([0 1 1 0],[0 0 1 1],c1);patch([0 1 1 1-e 1-e 0+e],[0 0 1 1-e 0+e 0+e],c2);patch([0 0 1 1-e 0+e 0+e],[0 1 1 1-e 1-e 0+e],c3);plot([0 1 1 0 0],[0 0 1 1 0]);disp('weights');
  "IW{2,1}(85,:)'" : Constant  Value=[-0.08772423791007770421668254812175291590392589569091796875;1.0195030887974543265528382107731886208057403564453125;-0.07897433955770442881583193184269475750625133514404296875;-0.06509672265964561166384783064131624996662139892578125;-1.78788283538337022804398657171986997127532958984375;-1.827232448706157530438076719292439520359039306640625;-1.4700634815470048355479093515896238386631011962890625;1.286243402850308914509014357463456690311431884765625]
      mask Display: e = 0.06;c1 = [120 150 230]/255;c2 = ([120 150 230]+0)/383;c3 = ([120 150 230]+128)/383;patch([0 1 1 0],[0 0 1 1],c1);patch([0 1 1 1-e 1-e 0+e],[0 0 1 1-e 0+e 0+e],c2);patch([0 0 1 1-e 0+e 0+e],[0 1 1 1-e 1-e 0+e],c3);plot([0 1 1 0 0],[0 0 1 1 0]);disp('weights');
  "IW{2,1}(850,:)'" : Constant  Value=[-1.2568053963437113562662261756486259400844573974609375;1.9016823511563523130263320126687176525592803955078125;0.058671608851267265105633441635291092097759246826171875;-1.2663658421639443218964515835978090763092041015625;0.10180163606827818956190867538680322468280792236328125;-0.282077878186899166923495840819668956100940704345703125;-1.17555827015038705241067873430438339710235595703125;1.6578784665706276513219563639722764492034912109375]
      mask Display: e = 0.06;c1 = [120 150 230]/255;c2 = ([120 150 230]+0)/383;c3 = ([120 150 230]+128)/383;patch([0 1 1 0],[0 0 1 1],c1);patch([0 1 1 1-e 1-e 0+e],[0 0 1 1-e 0+e 0+e],c2);patch([0 0 1 1-e 0+e 0+e],[0 1 1 1-e 1-e 0+e],c3);plot([0 1 1 0 0],[0 0 1 1 0]);disp('weights');
  "IW{2,1}(851,:)'" : Constant  Value=[0.568500387922301175791517380275763571262359619140625;1.6920693784728546571471952120191417634487152099609375;-1.8389914724546982949249240846256725490093231201171875;0.0279357810084018935714578191209511714987456798553466796875;0.3837477647992229012885445627034641802310943603515625;2.0501629532885576878697975189425051212310791015625;0.29185113398233963888372954897931776940822601318359375;-0.088612355321473212921290496524306945502758026123046875]
      mask Display: e = 0.06;c1 = [120 150 230]/255;c2 = ([120 150 230]+0)/383;c3 = ([120 150 230]+128)/383;patch([0 1 1 0],[0 0 1 1],c1);patch([0 1 1 1-e 1-e 0+e],[0 0 1 1-e 0+e 0+e],c2);patch([0 0 1 1-e 0+e 0+e],[0 1 1 1-e 1-e 0+e],c3);plot([0 1 1 0 0],[0 0 1 1 0]);disp('weights');
  "IW{2,1}(852,:)'" : Constant  Value=[-1.0959225090307687100477096464601345360279083251953125;-1.302468684089542083626156454556621611118316650390625;0.8162657522646223906548357263091020286083221435546875;-0.6329147713671068320451240651891566812992095947265625;-1.1326135259371330477051742491312325000762939453125;-0.07930619360205266865637696582780336029827594757080078125;-1.5153055972721138910941363064921461045742034912109375;1.865530950718959690703968590241856873035430908203125]
      mask Display: e = 0.06;c1 = [120 150 230]/255;c2 = ([120 150 230]+0)/383;c3 = ([120 150 230]+128)/383;patch([0 1 1 0],[0 0 1 1],c1);patch([0 1 1 1-e 1-e 0+e],[0 0 1 1-e 0+e 0+e],c2);patch([0 0 1 1-e 0+e 0+e],[0 1 1 1-e 1-e 0+e],c3);plot([0 1 1 0 0],[0 0 1 1 0]);disp('weights');
  "IW{2,1}(853,:)'" : Constant  Value=[2.04059306830559084033893668674863874912261962890625;1.09191275861406378311357912025414407253265380859375;0.1328954698551868818245935699451365508139133453369140625;0.911557667869038024122119168168865144252777099609375;0.053778568231589052306418352600303478538990020751953125;-2.065338637503702390318949255743063986301422119140625;0.4992965950357477478149803573614917695522308349609375;0.54568518687457989724265416953130625188350677490234375]
      mask Display: e = 0.06;c1 = [120 150 230]/255;c2 = ([120 150 230]+0)/383;c3 = ([120 150 230]+128)/383;patch([0 1 1 0],[0 0 1 1],c1);patch([0 1 1 1-e 1-e 0+e],[0 0 1 1-e 0+e 0+e],c2);patch([0 0 1 1-e 0+e 0+e],[0 1 1 1-e 1-e 0+e],c3);plot([0 1 1 0 0],[0 0 1 1 0]);disp('weights');
  "IW{2,1}(854,:)'" : Constant  Value=[1.7232420990767043367242195017752237617969512939453125;-1.7472972846092684751084789240849204361438751220703125;-0.229063125724689398143851803979487158358097076416015625;-1.889904469948759047071007444174028933048248291015625;-0.8010754430008308890620583042618818581104278564453125;0.99262681270497876706571105387411080300807952880859375;0.12381341956756582167731295385237899608910083770751953125;0.0021970371355703025885441892484095660620369017124176025390625]
      mask Display: e = 0.06;c1 = [120 150 230]/255;c2 = ([120 150 230]+0)/383;c3 = ([120 150 230]+128)/383;patch([0 1 1 0],[0 0 1 1],c1);patch([0 1 1 1-e 1-e 0+e],[0 0 1 1-e 0+e 0+e],c2);patch([0 0 1 1-e 0+e 0+e],[0 1 1 1-e 1-e 0+e],c3);plot([0 1 1 0 0],[0 0 1 1 0]);disp('weights');
  "IW{2,1}(855,:)'" : Constant  Value=[1.2241998405105871672304829189670272171497344970703125;-0.099717909171681273772236409058677963912487030029296875;-1.3548771133449009074212199266185052692890167236328125;1.31554683948929973524855085997842252254486083984375;-0.346061006639271084850406623445451259613037109375;-1.6418690584299884260843782612937502562999725341796875;-0.08911405353510039317743718356723547913134098052978515625;1.748153550898765562493508696206845343112945556640625]
      mask Display: e = 0.06;c1 = [120 150 230]/255;c2 = ([120 150 230]+0)/383;c3 = ([120 150 230]+128)/383;patch([0 1 1 0],[0 0 1 1],c1);patch([0 1 1 1-e 1-e 0+e],[0 0 1 1-e 0+e 0+e],c2);patch([0 0 1 1-e 0+e 0+e],[0 1 1 1-e 1-e 0+e],c3);plot([0 1 1 0 0],[0 0 1 1 0]);disp('weights');
  "IW{2,1}(856,:)'" : Constant  Value=[0.464415708685900041619021294536651112139225006103515625;1.623450577227948610214980362798087298870086669921875;1.32594336132155721230674316757358610630035400390625;1.622589827898302861086676784907467663288116455078125;-0.9773545894052186877587473645689897239208221435546875;0.9148205981002213160735436758841387927532196044921875;-0.310687479501002783432994647228042595088481903076171875;1.378188147670517338383433525450527667999267578125]
      mask Display: e = 0.06;c1 = [120 150 230]/255;c2 = ([120 150 230]+0)/383;c3 = ([120 150 230]+128)/383;patch([0 1 1 0],[0 0 1 1],c1);patch([0 1 1 1-e 1-e 0+e],[0 0 1 1-e 0+e 0+e],c2);patch([0 0 1 1-e 0+e 0+e],[0 1 1 1-e 1-e 0+e],c3);plot([0 1 1 0 0],[0 0 1 1 0]);disp('weights');
  "IW{2,1}(857,:)'" : Constant  Value=[1.508990515076394256510639024781994521617889404296875;-0.75336261994528752605759791549644432961940765380859375;-0.78739978359735862678547846371657215058803558349609375;-1.1445632897005693084935273873270489275455474853515625;-0.11988118104818125397859063241412513889372348785400390625;1.1162592752906179693894728188752196729183197021484375;-1.2940505370032229226495701368548907339572906494140625;-1.745552048269505718280925066210329532623291015625]
      mask Display: e = 0.06;c1 = [120 150 230]/255;c2 = ([120 150 230]+0)/383;c3 = ([120 150 230]+128)/383;patch([0 1 1 0],[0 0 1 1],c1);patch([0 1 1 1-e 1-e 0+e],[0 0 1 1-e 0+e 0+e],c2);patch([0 0 1 1-e 0+e 0+e],[0 1 1 1-e 1-e 0+e],c3);plot([0 1 1 0 0],[0 0 1 1 0]);disp('weights');
  "IW{2,1}(858,:)'" : Constant  Value=[-0.1813836428497411501492564411819330416619777679443359375;-1.4825108189725464402641819106065668165683746337890625;0.74943642098882323754338585786172188818454742431640625;-0.86222089672193902298857892674277536571025848388671875;-1.577600179805411340083765026065520942211151123046875;1.8195318302294058998569425966707058250904083251953125;0.037704355628558304525110855820457800291478633880615234375;-1.298029832441506936646646863664500415325164794921875]
      mask Display: e = 0.06;c1 = [120 150 230]/255;c2 = ([120 150 230]+0)/383;c3 = ([120 150 230]+128)/383;patch([0 1 1 0],[0 0 1 1],c1);patch([0 1 1 1-e 1-e 0+e],[0 0 1 1-e 0+e 0+e],c2);patch([0 0 1 1-e 0+e 0+e],[0 1 1 1-e 1-e 0+e],c3);plot([0 1 1 0 0],[0 0 1 1 0]);disp('weights');
  "IW{2,1}(859,:)'" : Constant  Value=[0.6582804541527706998493840728770010173320770263671875;1.1060246491057028617177593332598917186260223388671875;-1.740788394391317606135771711706183850765228271484375;1.13011562995246084284417520393617451190948486328125;-1.890025386330989487504439239273779094219207763671875;0.32080769119301943970157253716024570167064666748046875;-0.9349376438025160940270552600850351154804229736328125;-0.5359032983507090452945931247086264193058013916015625]
      mask Display: e = 0.06;c1 = [120 150 230]/255;c2 = ([120 150 230]+0)/383;c3 = ([120 150 230]+128)/383;patch([0 1 1 0],[0 0 1 1],c1);patch([0 1 1 1-e 1-e 0+e],[0 0 1 1-e 0+e 0+e],c2);patch([0 0 1 1-e 0+e 0+e],[0 1 1 1-e 1-e 0+e],c3);plot([0 1 1 0 0],[0 0 1 1 0]);disp('weights');
  "IW{2,1}(86,:)'" : Constant  Value=[-1.4037625566692526479783964532543905079364776611328125;2.640120196541260622069557939539663493633270263671875;-0.057447217397055071186340313715845695696771144866943359375;1.0900769534537386729056152034900151193141937255859375;0.64147920248788159458541713320300914347171783447265625;-0.0002258406805465892354910228956299533820128999650478363037109375;-0.5091962455457375025247301891795359551906585693359375;-0.460597098914463931595975054733571596443653106689453125]
      mask Display: e = 0.06;c1 = [120 150 230]/255;c2 = ([120 150 230]+0)/383;c3 = ([120 150 230]+128)/383;patch([0 1 1 0],[0 0 1 1],c1);patch([0 1 1 1-e 1-e 0+e],[0 0 1 1-e 0+e 0+e],c2);patch([0 0 1 1-e 0+e 0+e],[0 1 1 1-e 1-e 0+e],c3);plot([0 1 1 0 0],[0 0 1 1 0]);disp('weights');
  "IW{2,1}(860,:)'" : Constant  Value=[-1.574631394567351794222531680134125053882598876953125;1.0944347204656192928950986242853105068206787109375;-0.75883743431389250044816208173870109021663665771484375;1.6094929086046725341674346054787747561931610107421875;-1.381990246765451235688715314608998596668243408203125;-0.96570012344273992166421294314204715192317962646484375;0.97837329811756268416189641357050277292728424072265625;0.6011632959286734578796540517942048609256744384765625]
      mask Display: e = 0.06;c1 = [120 150 230]/255;c2 = ([120 150 230]+0)/383;c3 = ([120 150 230]+128)/383;patch([0 1 1 0],[0 0 1 1],c1);patch([0 1 1 1-e 1-e 0+e],[0 0 1 1-e 0+e 0+e],c2);patch([0 0 1 1-e 0+e 0+e],[0 1 1 1-e 1-e 0+e],c3);plot([0 1 1 0 0],[0 0 1 1 0]);disp('weights');
  "IW{2,1}(861,:)'" : Constant  Value=[-1.5748325733797603476205040351487696170806884765625;1.5616824643907116776375687550171278417110443115234375;1.1799693497673329201091974027804099023342132568359375;0.057407601352260133331650848731442238204181194305419921875;-0.5253802302925139056100078960298560559749603271484375;1.46824570370830542742623947560787200927734375;-0.2319682865641765345809943710264633409678936004638671875;-1.48720625632535075055784545838832855224609375]
      mask Display: e = 0.06;c1 = [120 150 230]/255;c2 = ([120 150 230]+0)/383;c3 = ([120 150 230]+128)/383;patch([0 1 1 0],[0 0 1 1],c1);patch([0 1 1 1-e 1-e 0+e],[0 0 1 1-e 0+e 0+e],c2);patch([0 0 1 1-e 0+e 0+e],[0 1 1 1-e 1-e 0+e],c3);plot([0 1 1 0 0],[0 0 1 1 0]);disp('weights');
  "IW{2,1}(862,:)'" : Constant  Value=[-1.607100070357324828052014709101058542728424072265625;-1.099409956949583655472224563709460198879241943359375;-1.1775681888025706367528755436069332063198089599609375;-1.608595885959430038525397321791388094425201416015625;-1.147362697990470525866157913696952164173126220703125;0.992735559593949101753196373465470969676971435546875;-0.979040297330556086308206431567668914794921875;0.06477713914980108567132077723726979456841945648193359375]
      mask Display: e = 0.06;c1 = [120 150 230]/255;c2 = ([120 150 230]+0)/383;c3 = ([120 150 230]+128)/383;patch([0 1 1 0],[0 0 1 1],c1);patch([0 1 1 1-e 1-e 0+e],[0 0 1 1-e 0+e 0+e],c2);patch([0 0 1 1-e 0+e 0+e],[0 1 1 1-e 1-e 0+e],c3);plot([0 1 1 0 0],[0 0 1 1 0]);disp('weights');
  "IW{2,1}(863,:)'" : Constant  Value=[1.016468179490713996671047425479628145694732666015625;-1.324418073754527913621359402895905077457427978515625;-1.9350799195729593282777614149381406605243682861328125;0.72360216564822199547535319652524776756763458251953125;0.260305435041020716280257829566835425794124603271484375;-0.71832174333938281218792099025449715554714202880859375;-1.7692932014929170225769894386758096516132354736328125;-0.318969541228806441335308363704825751483440399169921875]
      mask Display: e = 0.06;c1 = [120 150 230]/255;c2 = ([120 150 230]+0)/383;c3 = ([120 150 230]+128)/383;patch([0 1 1 0],[0 0 1 1],c1);patch([0 1 1 1-e 1-e 0+e],[0 0 1 1-e 0+e 0+e],c2);patch([0 0 1 1-e 0+e 0+e],[0 1 1 1-e 1-e 0+e],c3);plot([0 1 1 0 0],[0 0 1 1 0]);disp('weights');
  "IW{2,1}(864,:)'" : Constant  Value=[1.228244201446034633562476301449351012706756591796875;-1.105007442543133766577057031099684536457061767578125;0.917628854614623623575653255102224647998809814453125;0.8224886455236311011418592897825874388217926025390625;-1.0050508967524021119999133588862605392932891845703125;-0.6514231450128027400836572269327007234096527099609375;1.932653885867765541917151494999416172504425048828125;1.2659490343284012237035085490788333117961883544921875]
      mask Display: e = 0.06;c1 = [120 150 230]/255;c2 = ([120 150 230]+0)/383;c3 = ([120 150 230]+128)/383;patch([0 1 1 0],[0 0 1 1],c1);patch([0 1 1 1-e 1-e 0+e],[0 0 1 1-e 0+e 0+e],c2);patch([0 0 1 1-e 0+e 0+e],[0 1 1 1-e 1-e 0+e],c3);plot([0 1 1 0 0],[0 0 1 1 0]);disp('weights');
  "IW{2,1}(865,:)'" : Constant  Value=[1.2056517875902879044502924443804658949375152587890625;-1.0295805159679292106744696866371668875217437744140625;0.1998538336253029290556781916166073642671108245849609375;-0.83054548570240138705145227504544891417026519775390625;1.184117032186737805687926083919592201709747314453125;-0.77582849622791327792725724066258408129215240478515625;1.5924804763011264352456919368705712258815765380859375;-1.7888869731069114710209078111802227795124053955078125]
      mask Display: e = 0.06;c1 = [120 150 230]/255;c2 = ([120 150 230]+0)/383;c3 = ([120 150 230]+128)/383;patch([0 1 1 0],[0 0 1 1],c1);patch([0 1 1 1-e 1-e 0+e],[0 0 1 1-e 0+e 0+e],c2);patch([0 0 1 1-e 0+e 0+e],[0 1 1 1-e 1-e 0+e],c3);plot([0 1 1 0 0],[0 0 1 1 0]);disp('weights');
  "IW{2,1}(866,:)'" : Constant  Value=[-0.5134789135191575315531054002349264919757843017578125;-0.364008585968651543485208321726531721651554107666015625;-1.5503492507806948541571046007447876036167144775390625;-1.164320971426659578895623781136237084865570068359375;0.16564782764294327943588314155931584537029266357421875;1.1731804922252713208052909976686351001262664794921875;1.9762233192783436042105904562049545347690582275390625;-1.2412983020360839336859726245165802538394927978515625]
      mask Display: e = 0.06;c1 = [120 150 230]/255;c2 = ([120 150 230]+0)/383;c3 = ([120 150 230]+128)/383;patch([0 1 1 0],[0 0 1 1],c1);patch([0 1 1 1-e 1-e 0+e],[0 0 1 1-e 0+e 0+e],c2);patch([0 0 1 1-e 0+e 0+e],[0 1 1 1-e 1-e 0+e],c3);plot([0 1 1 0 0],[0 0 1 1 0]);disp('weights');
  "IW{2,1}(867,:)'" : Constant  Value=[-1.3313511081139584035781808779574930667877197265625;-0.43702393869276023874448355854838155210018157958984375;-1.02405240800845209747649278142489492893218994140625;0.7049266971999321729214216247783042490482330322265625;0.9294343197212970864029557560570538043975830078125;1.03801700495555149217352663981728255748748779296875;1.9600062237774835693926434032618999481201171875;1.29436532002251514228419182472862303256988525390625]
      mask Display: e = 0.06;c1 = [120 150 230]/255;c2 = ([120 150 230]+0)/383;c3 = ([120 150 230]+128)/383;patch([0 1 1 0],[0 0 1 1],c1);patch([0 1 1 1-e 1-e 0+e],[0 0 1 1-e 0+e 0+e],c2);patch([0 0 1 1-e 0+e 0+e],[0 1 1 1-e 1-e 0+e],c3);plot([0 1 1 0 0],[0 0 1 1 0]);disp('weights');
  "IW{2,1}(868,:)'" : Constant  Value=[-0.02493792271422150264026385002580354921519756317138671875;-2.113756054606455325739489126135595142841339111328125;0.08185241112456055623258777131923125125467777252197265625;-1.6140363809951698836897548972046934068202972412109375;-0.70732835224402013096778318868018686771392822265625;1.2524288838514825439318656208342872560024261474609375;-1.070842227112267064370598745881579816341400146484375;-0.85471433683648034840274476664490066468715667724609375]
      mask Display: e = 0.06;c1 = [120 150 230]/255;c2 = ([120 150 230]+0)/383;c3 = ([120 150 230]+128)/383;patch([0 1 1 0],[0 0 1 1],c1);patch([0 1 1 1-e 1-e 0+e],[0 0 1 1-e 0+e 0+e],c2);patch([0 0 1 1-e 0+e 0+e],[0 1 1 1-e 1-e 0+e],c3);plot([0 1 1 0 0],[0 0 1 1 0]);disp('weights');
  "IW{2,1}(869,:)'" : Constant  Value=[-1.54689869752372910483018131344579160213470458984375;-0.72364963009258109760679644750780425965785980224609375;-0.442099894501953027958762731941533274948596954345703125;1.2718595081469334928669923101551830768585205078125;1.291395836788753914703420377918519079685211181640625;0.91812630632145941778077258277335204184055328369140625;1.4679586549886443069823371843085624277591705322265625;-1.28532694351242238184340749285183846950531005859375]
      mask Display: e = 0.06;c1 = [120 150 230]/255;c2 = ([120 150 230]+0)/383;c3 = ([120 150 230]+128)/383;patch([0 1 1 0],[0 0 1 1],c1);patch([0 1 1 1-e 1-e 0+e],[0 0 1 1-e 0+e 0+e],c2);patch([0 0 1 1-e 0+e 0+e],[0 1 1 1-e 1-e 0+e],c3);plot([0 1 1 0 0],[0 0 1 1 0]);disp('weights');
  "IW{2,1}(87,:)'" : Constant  Value=[-1.2528917637200176482537017363938502967357635498046875;1.5172456390287809568917509750463068485260009765625;1.1512757567676528136502156485221348702907562255859375;-1.4105101402828619239215868219616822898387908935546875;-1.5153385475840435159256003316841088235378265380859375;0.6502799980283653358270612443448044359683990478515625;0.55581507677277619539069064558134414255619049072265625;-0.80290832175172222040515634944313205778598785400390625]
      mask Display: e = 0.06;c1 = [120 150 230]/255;c2 = ([120 150 230]+0)/383;c3 = ([120 150 230]+128)/383;patch([0 1 1 0],[0 0 1 1],c1);patch([0 1 1 1-e 1-e 0+e],[0 0 1 1-e 0+e 0+e],c2);patch([0 0 1 1-e 0+e 0+e],[0 1 1 1-e 1-e 0+e],c3);plot([0 1 1 0 0],[0 0 1 1 0]);disp('weights');
  "IW{2,1}(870,:)'" : Constant  Value=[-1.3689807432850045199046462585101835429668426513671875;1.59777988801387937911613335018046200275421142578125;-1.4658684623222999476865879842080175876617431640625;1.62528380872843758453427653876133263111114501953125;-0.038116693315516515794261209748583496548235416412353515625;0.10209888033702395337964929922236478887498378753662109375;-0.58417029517840146635165865518501959741115570068359375;1.2774430979464312940763193182647228240966796875]
      mask Display: e = 0.06;c1 = [120 150 230]/255;c2 = ([120 150 230]+0)/383;c3 = ([120 150 230]+128)/383;patch([0 1 1 0],[0 0 1 1],c1);patch([0 1 1 1-e 1-e 0+e],[0 0 1 1-e 0+e 0+e],c2);patch([0 0 1 1-e 0+e 0+e],[0 1 1 1-e 1-e 0+e],c3);plot([0 1 1 0 0],[0 0 1 1 0]);disp('weights');
  "IW{2,1}(871,:)'" : Constant  Value=[-1.2900360118187912394915883851354010403156280517578125;1.6165110669254370012737354045384563505649566650390625;-1.741634579560183748725421537528745830059051513671875;0.76815999794583678106363322513061575591564178466796875;0.2717717814424827071917434295755811035633087158203125;0.1432616094128208172886473903417936526238918304443359375;0.10016508079632123473512450573252863250672817230224609375;-1.7431129797125068936480829506763257086277008056640625]
      mask Display: e = 0.06;c1 = [120 150 230]/255;c2 = ([120 150 230]+0)/383;c3 = ([120 150 230]+128)/383;patch([0 1 1 0],[0 0 1 1],c1);patch([0 1 1 1-e 1-e 0+e],[0 0 1 1-e 0+e 0+e],c2);patch([0 0 1 1-e 0+e 0+e],[0 1 1 1-e 1-e 0+e],c3);plot([0 1 1 0 0],[0 0 1 1 0]);disp('weights');
  "IW{2,1}(872,:)'" : Constant  Value=[0.09243712238496504252083241226500831544399261474609375;-1.5984255200472838875924708190723322331905364990234375;-1.305778479234344313653082281234674155712127685546875;-0.65902899499126998961173740099184215068817138671875;-0.996898430668823554157143007614649832248687744140625;-1.5892518032102860292553714316454716026782989501953125;1.305161706952731481834462101687677204608917236328125;-1.1174836145302309287075104293762706220149993896484375]
      mask Display: e = 0.06;c1 = [120 150 230]/255;c2 = ([120 150 230]+0)/383;c3 = ([120 150 230]+128)/383;patch([0 1 1 0],[0 0 1 1],c1);patch([0 1 1 1-e 1-e 0+e],[0 0 1 1-e 0+e 0+e],c2);patch([0 0 1 1-e 0+e 0+e],[0 1 1 1-e 1-e 0+e],c3);plot([0 1 1 0 0],[0 0 1 1 0]);disp('weights');
  "IW{2,1}(873,:)'" : Constant  Value=[1.216642750432074482347388766356743872165679931640625;0.6821327292441019540802926712785847485065460205078125;-1.6971631898610606281607715573045425117015838623046875;0.327572923803334636883022312758839689195156097412109375;1.16247481813381181581235068733803927898406982421875;1.4878364450885677161551257086102850735187530517578125;0.032923476006438433250078645642133778892457485198974609375;1.5929199039957959715962942937039770185947418212890625]
      mask Display: e = 0.06;c1 = [120 150 230]/255;c2 = ([120 150 230]+0)/383;c3 = ([120 150 230]+128)/383;patch([0 1 1 0],[0 0 1 1],c1);patch([0 1 1 1-e 1-e 0+e],[0 0 1 1-e 0+e 0+e],c2);patch([0 0 1 1-e 0+e 0+e],[0 1 1 1-e 1-e 0+e],c3);plot([0 1 1 0 0],[0 0 1 1 0]);disp('weights');
  "IW{2,1}(874,:)'" : Constant  Value=[1.306598601303817108743032804341055452823638916015625;0.61044882164419178582903668939252384006977081298828125;-1.5109751413581735679514395087608136236667633056640625;-1.50483109197571796045167502597905695438385009765625;1.0172080178450284559943384010693989694118499755859375;-0.5216190218056449001693408717983402311801910400390625;-1.3756976449050337674151478495332412421703338623046875;1.195680999285163803591558462358079850673675537109375]
      mask Display: e = 0.06;c1 = [120 150 230]/255;c2 = ([120 150 230]+0)/383;c3 = ([120 150 230]+128)/383;patch([0 1 1 0],[0 0 1 1],c1);patch([0 1 1 1-e 1-e 0+e],[0 0 1 1-e 0+e 0+e],c2);patch([0 0 1 1-e 0+e 0+e],[0 1 1 1-e 1-e 0+e],c3);plot([0 1 1 0 0],[0 0 1 1 0]);disp('weights');
  "IW{2,1}(875,:)'" : Constant  Value=[1.4721307499040110489119115300127305090427398681640625;1.541647953950369132058995091938413679599761962890625;1.231406031886434160327326026163063943386077880859375;-1.5057615482835349229873145304736681282520294189453125;-0.87308136996386387362889536234433762729167938232421875;0.58708912125710355223162650872836820781230926513671875;-0.3609455879835932190502489902428351342678070068359375;1.203036226912870265692845350713469088077545166015625]
      mask Display: e = 0.06;c1 = [120 150 230]/255;c2 = ([120 150 230]+0)/383;c3 = ([120 150 230]+128)/383;patch([0 1 1 0],[0 0 1 1],c1);patch([0 1 1 1-e 1-e 0+e],[0 0 1 1-e 0+e 0+e],c2);patch([0 0 1 1-e 0+e 0+e],[0 1 1 1-e 1-e 0+e],c3);plot([0 1 1 0 0],[0 0 1 1 0]);disp('weights');
  "IW{2,1}(876,:)'" : Constant  Value=[-1.168014045577878246007230700342915952205657958984375;0.6751044224139242100335422946955077350139617919921875;1.7882880942725523087943884092965163290500640869140625;1.5766599291758061074375518728629685938358306884765625;-0.0170079933024334280233791361069961567409336566925048828125;-0.9122092698736803395576089314999990165233612060546875;0.275138579200516153466793412007973529398441314697265625;1.6965882410401358360019230531179346144199371337890625]
      mask Display: e = 0.06;c1 = [120 150 230]/255;c2 = ([120 150 230]+0)/383;c3 = ([120 150 230]+128)/383;patch([0 1 1 0],[0 0 1 1],c1);patch([0 1 1 1-e 1-e 0+e],[0 0 1 1-e 0+e 0+e],c2);patch([0 0 1 1-e 0+e 0+e],[0 1 1 1-e 1-e 0+e],c3);plot([0 1 1 0 0],[0 0 1 1 0]);disp('weights');
  "IW{2,1}(877,:)'" : Constant  Value=[1.227547394728553786791280799661763012409210205078125;-0.28520510797059783758555795429856516420841217041015625;-1.2309944020338281500670518653350882232189178466796875;0.381049657679092212969607089689816348254680633544921875;0.041656961304828050984827569891422172077000141143798828125;1.813586326983581020755309509695507586002349853515625;1.1349593144340222039545551524497568607330322265625;1.7855234840570559651240500897984020411968231201171875]
      mask Display: e = 0.06;c1 = [120 150 230]/255;c2 = ([120 150 230]+0)/383;c3 = ([120 150 230]+128)/383;patch([0 1 1 0],[0 0 1 1],c1);patch([0 1 1 1-e 1-e 0+e],[0 0 1 1-e 0+e 0+e],c2);patch([0 0 1 1-e 0+e 0+e],[0 1 1 1-e 1-e 0+e],c3);plot([0 1 1 0 0],[0 0 1 1 0]);disp('weights');
  "IW{2,1}(878,:)'" : Constant  Value=[0.478491456800045844577340403702692128717899322509765625;-1.603225632819123003258710014051757752895355224609375;1.5450523780938476559043692759587429463863372802734375;0.08559822985565897213167119161880691535770893096923828125;1.63201044891770319367196862003766000270843505859375;0.04147376500642148411390763840245199389755725860595703125;1.02440104371904272539950397913344204425811767578125;-1.4511209729142755531228203835780732333660125732421875]
      mask Display: e = 0.06;c1 = [120 150 230]/255;c2 = ([120 150 230]+0)/383;c3 = ([120 150 230]+128)/383;patch([0 1 1 0],[0 0 1 1],c1);patch([0 1 1 1-e 1-e 0+e],[0 0 1 1-e 0+e 0+e],c2);patch([0 0 1 1-e 0+e 0+e],[0 1 1 1-e 1-e 0+e],c3);plot([0 1 1 0 0],[0 0 1 1 0]);disp('weights');
  "IW{2,1}(879,:)'" : Constant  Value=[1.1452375318430225714649850488058291375637054443359375;-0.89557375605331379642137790142442099750041961669921875;-1.333172286600245559640143255819566547870635986328125;-1.4501736299530474383345790556631982326507568359375;-0.421844354397880760831895941009861417114734649658203125;1.518649713059658790115236115525476634502410888671875;0.25117898857968257164685610405285842716693878173828125;-1.489326407103693572508973375079222023487091064453125]
      mask Display: e = 0.06;c1 = [120 150 230]/255;c2 = ([120 150 230]+0)/383;c3 = ([120 150 230]+128)/383;patch([0 1 1 0],[0 0 1 1],c1);patch([0 1 1 1-e 1-e 0+e],[0 0 1 1-e 0+e 0+e],c2);patch([0 0 1 1-e 0+e 0+e],[0 1 1 1-e 1-e 0+e],c3);plot([0 1 1 0 0],[0 0 1 1 0]);disp('weights');
  "IW{2,1}(88,:)'" : Constant  Value=[-1.6649362484104910375748431761167012155055999755859375;-1.410140347241286118418202022439800202846527099609375;1.0097091271972435944093149373657070100307464599609375;-0.8642372305862180414948170437128283083438873291015625;-0.625799756920939476145804292173124849796295166015625;-0.251354895029050673382897684859926812350749969482421875;0.0187522411894114338082317772204987704753875732421875;2.06270751681129382859580800868570804595947265625]
      mask Display: e = 0.06;c1 = [120 150 230]/255;c2 = ([120 150 230]+0)/383;c3 = ([120 150 230]+128)/383;patch([0 1 1 0],[0 0 1 1],c1);patch([0 1 1 1-e 1-e 0+e],[0 0 1 1-e 0+e 0+e],c2);patch([0 0 1 1-e 0+e 0+e],[0 1 1 1-e 1-e 0+e],c3);plot([0 1 1 0 0],[0 0 1 1 0]);disp('weights');
  "IW{2,1}(880,:)'" : Constant  Value=[-1.5113677489113401808396019987412728369235992431640625;-0.51496536873876552764528469197102822363376617431640625;1.3450256548560519664903267766931094229221343994140625;-1.4753715803622065028122278818045742809772491455078125;0.2289429929225571258566418464397429488599300384521484375;0.822610042192525536819402987021021544933319091796875;0.6514678074571091936917355269542895257472991943359375;-1.8300970966359793035138636696501635015010833740234375]
      mask Display: e = 0.06;c1 = [120 150 230]/255;c2 = ([120 150 230]+0)/383;c3 = ([120 150 230]+128)/383;patch([0 1 1 0],[0 0 1 1],c1);patch([0 1 1 1-e 1-e 0+e],[0 0 1 1-e 0+e 0+e],c2);patch([0 0 1 1-e 0+e 0+e],[0 1 1 1-e 1-e 0+e],c3);plot([0 1 1 0 0],[0 0 1 1 0]);disp('weights');
  "IW{2,1}(881,:)'" : Constant  Value=[1.6133311303259632030204784314264543354511260986328125;-0.051675826680349278008375080162295489571988582611083984375;-0.7383697205156440901419045985676348209381103515625;-1.58574821635733087532571516931056976318359375;-1.5300555878679988897062003161408938467502593994140625;-0.7264637976078731629314688689191825687885284423828125;-0.93652875037203331398671934948652051389217376708984375;-1.3053557436361433730098724481649696826934814453125]
      mask Display: e = 0.06;c1 = [120 150 230]/255;c2 = ([120 150 230]+0)/383;c3 = ([120 150 230]+128)/383;patch([0 1 1 0],[0 0 1 1],c1);patch([0 1 1 1-e 1-e 0+e],[0 0 1 1-e 0+e 0+e],c2);patch([0 0 1 1-e 0+e 0+e],[0 1 1 1-e 1-e 0+e],c3);plot([0 1 1 0 0],[0 0 1 1 0]);disp('weights');
  "IW{2,1}(882,:)'" : Constant  Value=[-1.3886823286690608281190861816867254674434661865234375;1.5553148798007694342260265329969115555286407470703125;0.53457511204626040335341485842945985496044158935546875;-0.1313417199272401136855847880724468268454074859619140625;1.4843620947712843349819422655855305492877960205078125;1.215823867464832286344744716188870370388031005859375;0.09751089534952150916780055922572501003742218017578125;1.5429257305201005134875913427094928920269012451171875]
      mask Display: e = 0.06;c1 = [120 150 230]/255;c2 = ([120 150 230]+0)/383;c3 = ([120 150 230]+128)/383;patch([0 1 1 0],[0 0 1 1],c1);patch([0 1 1 1-e 1-e 0+e],[0 0 1 1-e 0+e 0+e],c2);patch([0 0 1 1-e 0+e 0+e],[0 1 1 1-e 1-e 0+e],c3);plot([0 1 1 0 0],[0 0 1 1 0]);disp('weights');
  "IW{2,1}(883,:)'" : Constant  Value=[0.02888150154797698709874254063834086991846561431884765625;-1.5006889530465847837348292159731499850749969482421875;-1.831474414774731496180493195424787700176239013671875;0.799353619353031508154572293278761208057403564453125;0.47134849150807145434782796655781567096710205078125;-0.61446701120321922662270708315190859138965606689453125;0.2243648739702932826123316090161097235977649688720703125;-2.06872962462936360594767393195070326328277587890625]
      mask Display: e = 0.06;c1 = [120 150 230]/255;c2 = ([120 150 230]+0)/383;c3 = ([120 150 230]+128)/383;patch([0 1 1 0],[0 0 1 1],c1);patch([0 1 1 1-e 1-e 0+e],[0 0 1 1-e 0+e 0+e],c2);patch([0 0 1 1-e 0+e 0+e],[0 1 1 1-e 1-e 0+e],c3);plot([0 1 1 0 0],[0 0 1 1 0]);disp('weights');
  "IW{2,1}(884,:)'" : Constant  Value=[0.395070676897717520947850289303460158407688140869140625;-0.507313268220934698859991840436123311519622802734375;0.84581680234846057242492634031805209815502166748046875;0.76019963356321740288734645218937657773494720458984375;-1.409001395916046561751500121317803859710693359375;2.297124900987922213602132615051232278347015380859375;-1.3203527569315427481200231341063044965267181396484375;-0.58382866637559349687336407441762275993824005126953125]
      mask Display: e = 0.06;c1 = [120 150 230]/255;c2 = ([120 150 230]+0)/383;c3 = ([120 150 230]+128)/383;patch([0 1 1 0],[0 0 1 1],c1);patch([0 1 1 1-e 1-e 0+e],[0 0 1 1-e 0+e 0+e],c2);patch([0 0 1 1-e 0+e 0+e],[0 1 1 1-e 1-e 0+e],c3);plot([0 1 1 0 0],[0 0 1 1 0]);disp('weights');
  "IW{2,1}(885,:)'" : Constant  Value=[1.9935121400496214061348609902779571712017059326171875;-1.0509117528087241755230252238106913864612579345703125;-1.1248662118409231691629202032345347106456756591796875;1.514251756220497124871826599701307713985443115234375;-0.9055730849755609934703670660383068025112152099609375;0.9191703212061839156632458980311639606952667236328125;-0.2304689210091804552060779087696573697030544281005859375;-0.78669550401637466929827269268571399152278900146484375]
      mask Display: e = 0.06;c1 = [120 150 230]/255;c2 = ([120 150 230]+0)/383;c3 = ([120 150 230]+128)/383;patch([0 1 1 0],[0 0 1 1],c1);patch([0 1 1 1-e 1-e 0+e],[0 0 1 1-e 0+e 0+e],c2);patch([0 0 1 1-e 0+e 0+e],[0 1 1 1-e 1-e 0+e],c3);plot([0 1 1 0 0],[0 0 1 1 0]);disp('weights');
  "IW{2,1}(886,:)'" : Constant  Value=[0.9180211072200326061221176132676191627979278564453125;0.64103387592749572210237829494872130453586578369140625;1.89793828563388000674194699968211352825164794921875;1.78924289246732737268530399887822568416595458984375;-0.01228229960164627272700688109807742876000702381134033203125;-0.106376393875732333516026528741349466145038604736328125;-1.6125412519285984291883551122737117111682891845703125;-0.596727211982277960800047367229126393795013427734375]
      mask Display: e = 0.06;c1 = [120 150 230]/255;c2 = ([120 150 230]+0)/383;c3 = ([120 150 230]+128)/383;patch([0 1 1 0],[0 0 1 1],c1);patch([0 1 1 1-e 1-e 0+e],[0 0 1 1-e 0+e 0+e],c2);patch([0 0 1 1-e 0+e 0+e],[0 1 1 1-e 1-e 0+e],c3);plot([0 1 1 0 0],[0 0 1 1 0]);disp('weights');
  "IW{2,1}(887,:)'" : Constant  Value=[-1.755699962005433878431404082220979034900665283203125;1.1477779316009619758887083662557415664196014404296875;-0.348935425209843386173957924256683327257633209228515625;0.234750463096006445340435675461776554584503173828125;1.5049995342387685326457358314655721187591552734375;-1.0592330836254004733376632430008612573146820068359375;0.753767232517407403946663180249743163585662841796875;-1.5955619956430491246379688163870014250278472900390625]
      mask Display: e = 0.06;c1 = [120 150 230]/255;c2 = ([120 150 230]+0)/383;c3 = ([120 150 230]+128)/383;patch([0 1 1 0],[0 0 1 1],c1);patch([0 1 1 1-e 1-e 0+e],[0 0 1 1-e 0+e 0+e],c2);patch([0 0 1 1-e 0+e 0+e],[0 1 1 1-e 1-e 0+e],c3);plot([0 1 1 0 0],[0 0 1 1 0]);disp('weights');
  "IW{2,1}(888,:)'" : Constant  Value=[-1.2340466498819342433534984593279659748077392578125;-0.8957777867205825028662502518272958695888519287109375;-1.17022199909074497981009699287824332714080810546875;0.6114277794812024158233043635846115648746490478515625;-1.1828583703850583663808038181741721928119659423828125;-0.9694739088649295677413419980439357459545135498046875;2.069440443249854322260716799064539372920989990234375;0.5813813843888879784316259247134439647197723388671875]
      mask Display: e = 0.06;c1 = [120 150 230]/255;c2 = ([120 150 230]+0)/383;c3 = ([120 150 230]+128)/383;patch([0 1 1 0],[0 0 1 1],c1);patch([0 1 1 1-e 1-e 0+e],[0 0 1 1-e 0+e 0+e],c2);patch([0 0 1 1-e 0+e 0+e],[0 1 1 1-e 1-e 0+e],c3);plot([0 1 1 0 0],[0 0 1 1 0]);disp('weights');
  "IW{2,1}(889,:)'" : Constant  Value=[-1.035564153891570082777207062463276088237762451171875;-0.896116298364627805739246468874625861644744873046875;-0.940019334512694815231270695221610367298126220703125;-1.6147952106761935819889686172246001660823822021484375;-0.6348051135413090850789785690722055733203887939453125;-1.914909169831271906758729528519324958324432373046875;1.20549006443307415992194364662282168865203857421875;-0.3808870370422512419139593475847505033016204833984375]
      mask Display: e = 0.06;c1 = [120 150 230]/255;c2 = ([120 150 230]+0)/383;c3 = ([120 150 230]+128)/383;patch([0 1 1 0],[0 0 1 1],c1);patch([0 1 1 1-e 1-e 0+e],[0 0 1 1-e 0+e 0+e],c2);patch([0 0 1 1-e 0+e 0+e],[0 1 1 1-e 1-e 0+e],c3);plot([0 1 1 0 0],[0 0 1 1 0]);disp('weights');
  "IW{2,1}(89,:)'" : Constant  Value=[1.706726949529194126142783716204576194286346435546875;1.524786571647256838701878223218955099582672119140625;-0.468023077207215809636409176164306700229644775390625;-0.09075538763878866765910657932181493379175662994384765625;-0.1625482764260429424663101372061646543443202972412109375;1.521577811780408406860942704952321946620941162109375;-1.4437198872279937145179928847937844693660736083984375;1.1466800154583831616861289148801006376743316650390625]
      mask Display: e = 0.06;c1 = [120 150 230]/255;c2 = ([120 150 230]+0)/383;c3 = ([120 150 230]+128)/383;patch([0 1 1 0],[0 0 1 1],c1);patch([0 1 1 1-e 1-e 0+e],[0 0 1 1-e 0+e 0+e],c2);patch([0 0 1 1-e 0+e 0+e],[0 1 1 1-e 1-e 0+e],c3);plot([0 1 1 0 0],[0 0 1 1 0]);disp('weights');
  "IW{2,1}(890,:)'" : Constant  Value=[-1.7887273607305704814507407718338072299957275390625;0.350771918604118881912512506460188888013362884521484375;-1.676243095301467089797142762108705937862396240234375;0.04509229091783724385766873865577508695423603057861328125;-1.0140840354430926684159430806175805628299713134765625;0.76152484141032272813021108959219418466091156005859375;-1.7968273193759507488920235118712298572063446044921875;-0.2287199115552786266025719896788359619677066802978515625]
      mask Display: e = 0.06;c1 = [120 150 230]/255;c2 = ([120 150 230]+0)/383;c3 = ([120 150 230]+128)/383;patch([0 1 1 0],[0 0 1 1],c1);patch([0 1 1 1-e 1-e 0+e],[0 0 1 1-e 0+e 0+e],c2);patch([0 0 1 1-e 0+e 0+e],[0 1 1 1-e 1-e 0+e],c3);plot([0 1 1 0 0],[0 0 1 1 0]);disp('weights');
  "IW{2,1}(891,:)'" : Constant  Value=[-1.19352466782382915511107057682238519191741943359375;1.850778045135327953829573743860237300395965576171875;1.311790398431209592189361501368694007396697998046875;0.313426053856100395034189887155662290751934051513671875;0.71725374739746161623088482883758842945098876953125;-0.8768108658734579119453655948746018111705780029296875;-1.5542352551833051865770585209247656166553497314453125;-0.7298367409633603752894259741879068315029144287109375]
      mask Display: e = 0.06;c1 = [120 150 230]/255;c2 = ([120 150 230]+0)/383;c3 = ([120 150 230]+128)/383;patch([0 1 1 0],[0 0 1 1],c1);patch([0 1 1 1-e 1-e 0+e],[0 0 1 1-e 0+e 0+e],c2);patch([0 0 1 1-e 0+e 0+e],[0 1 1 1-e 1-e 0+e],c3);plot([0 1 1 0 0],[0 0 1 1 0]);disp('weights');
  "IW{2,1}(892,:)'" : Constant  Value=[-1.3686285862478426711419388084323145449161529541015625;-1.5526866592649444243079415173269808292388916015625;0.654551535596534339589425144367851316928863525390625;0.6969239217629195071168624053825624287128448486328125;-1.1059021305150213976276063476689159870147705078125;-1.1338499606120979734669163008220493793487548828125;-1.11147166438306843616601327084936201572418212890625;1.442385491697983912473546297405846416950225830078125]
      mask Display: e = 0.06;c1 = [120 150 230]/255;c2 = ([120 150 230]+0)/383;c3 = ([120 150 230]+128)/383;patch([0 1 1 0],[0 0 1 1],c1);patch([0 1 1 1-e 1-e 0+e],[0 0 1 1-e 0+e 0+e],c2);patch([0 0 1 1-e 0+e 0+e],[0 1 1 1-e 1-e 0+e],c3);plot([0 1 1 0 0],[0 0 1 1 0]);disp('weights');
  "IW{2,1}(893,:)'" : Constant  Value=[0.9550994026803165670713724466622807085514068603515625;1.587693972721158530703178257681429386138916015625;-0.334052563194295715209847230653394944965839385986328125;1.683671963762920054108462863950990140438079833984375;1.663276699759348442597683970234356820583343505859375;-0.2115164768938664341391131529235281050205230712890625;-1.3355849710573719502093581468216143548488616943359375;-0.1707455750385998005658194642819580622017383575439453125]
      mask Display: e = 0.06;c1 = [120 150 230]/255;c2 = ([120 150 230]+0)/383;c3 = ([120 150 230]+128)/383;patch([0 1 1 0],[0 0 1 1],c1);patch([0 1 1 1-e 1-e 0+e],[0 0 1 1-e 0+e 0+e],c2);patch([0 0 1 1-e 0+e 0+e],[0 1 1 1-e 1-e 0+e],c3);plot([0 1 1 0 0],[0 0 1 1 0]);disp('weights');
  "IW{2,1}(894,:)'" : Constant  Value=[1.86583017634069303625210523023270070552825927734375;-0.78958566758121684348026292354916222393512725830078125;1.4702657453450707070174985346966423094272613525390625;-0.229012504003866468327288430373300798237323760986328125;0.69864505244221486446321023322525434195995330810546875;-0.53453686841239178573204071653890423476696014404296875;1.8627074104480276783846193211502395570278167724609375;0.68079252704151915764896330074407160282135009765625]
      mask Display: e = 0.06;c1 = [120 150 230]/255;c2 = ([120 150 230]+0)/383;c3 = ([120 150 230]+128)/383;patch([0 1 1 0],[0 0 1 1],c1);patch([0 1 1 1-e 1-e 0+e],[0 0 1 1-e 0+e 0+e],c2);patch([0 0 1 1-e 0+e 0+e],[0 1 1 1-e 1-e 0+e],c3);plot([0 1 1 0 0],[0 0 1 1 0]);disp('weights');
  "IW{2,1}(895,:)'" : Constant  Value=[1.946097101775736692985674380906857550144195556640625;1.2332389049590843921322402820806019008159637451171875;0.824666546724245552724141816725023090839385986328125;1.821984457717930272480089115560986101627349853515625;-0.10422144613535881674248884110056678764522075653076171875;0.72886887563868463235650096976314671337604522705078125;0.52765933148677512942725797984167002141475677490234375;-0.94515462563348418001396566978655755519866943359375]
      mask Display: e = 0.06;c1 = [120 150 230]/255;c2 = ([120 150 230]+0)/383;c3 = ([120 150 230]+128)/383;patch([0 1 1 0],[0 0 1 1],c1);patch([0 1 1 1-e 1-e 0+e],[0 0 1 1-e 0+e 0+e],c2);patch([0 0 1 1-e 0+e 0+e],[0 1 1 1-e 1-e 0+e],c3);plot([0 1 1 0 0],[0 0 1 1 0]);disp('weights');
  "IW{2,1}(896,:)'" : Constant  Value=[-1.556091650971600071073908111429773271083831787109375;-1.53319608764086634522527674562297761440277099609375;-1.5406022812846391634167275697109289467334747314453125;-0.82168390588254214268459918457665480673313140869140625;0.85706096099886497352571268493193201720714569091796875;1.3636630325023630927461226747254841029644012451171875;0.432614352439674387795776056009344756603240966796875;0.64767410671838454572224463845486752688884735107421875]
      mask Display: e = 0.06;c1 = [120 150 230]/255;c2 = ([120 150 230]+0)/383;c3 = ([120 150 230]+128)/383;patch([0 1 1 0],[0 0 1 1],c1);patch([0 1 1 1-e 1-e 0+e],[0 0 1 1-e 0+e 0+e],c2);patch([0 0 1 1-e 0+e 0+e],[0 1 1 1-e 1-e 0+e],c3);plot([0 1 1 0 0],[0 0 1 1 0]);disp('weights');
  "IW{2,1}(897,:)'" : Constant  Value=[-1.3420185743261365818312924602651037275791168212890625;0.05228813391616016215124318478046916425228118896484375;-1.92218240516822103103322660899721086025238037109375;-0.75808035220247826924122591663035564124584197998046875;0.1842301408038846677328592704725451767444610595703125;0.358731954207666292600009683155803941190242767333984375;-1.9434208230569585129643428444978781044483184814453125;-1.0080046003530671594461409767973236739635467529296875]
      mask Display: e = 0.06;c1 = [120 150 230]/255;c2 = ([120 150 230]+0)/383;c3 = ([120 150 230]+128)/383;patch([0 1 1 0],[0 0 1 1],c1);patch([0 1 1 1-e 1-e 0+e],[0 0 1 1-e 0+e 0+e],c2);patch([0 0 1 1-e 0+e 0+e],[0 1 1 1-e 1-e 0+e],c3);plot([0 1 1 0 0],[0 0 1 1 0]);disp('weights');
  "IW{2,1}(898,:)'" : Constant  Value=[-1.2845426831266595346647818587371148169040679931640625;-2.06805337703919889236203744076192378997802734375;-0.2008373952944750850946320497314445674419403076171875;1.7714073220406179043351357904612086713314056396484375;-0.238209588679963835122777027208940126001834869384765625;-0.282059494769808793979137817586888559162616729736328125;0.92364189092199777686431616530171595513820648193359375;-0.95414745071818873878299882562714628875255584716796875]
      mask Display: e = 0.06;c1 = [120 150 230]/255;c2 = ([120 150 230]+0)/383;c3 = ([120 150 230]+128)/383;patch([0 1 1 0],[0 0 1 1],c1);patch([0 1 1 1-e 1-e 0+e],[0 0 1 1-e 0+e 0+e],c2);patch([0 0 1 1-e 0+e 0+e],[0 1 1 1-e 1-e 0+e],c3);plot([0 1 1 0 0],[0 0 1 1 0]);disp('weights');
  "IW{2,1}(899,:)'" : Constant  Value=[-0.65431637408863274618653349534724839031696319580078125;0.4366867007536832101521895310725085437297821044921875;1.931050278347616444563072946039028465747833251953125;-1.096327713187276398087988127372227609157562255859375;-1.6131652603499400111530803769710473716259002685546875;0.197454341454030235514238711402867920696735382080078125;-0.1505033716726986992018311184438061900436878204345703125;-1.677344723367415912917977038887329399585723876953125]
      mask Display: e = 0.06;c1 = [120 150 230]/255;c2 = ([120 150 230]+0)/383;c3 = ([120 150 230]+128)/383;patch([0 1 1 0],[0 0 1 1],c1);patch([0 1 1 1-e 1-e 0+e],[0 0 1 1-e 0+e 0+e],c2);patch([0 0 1 1-e 0+e 0+e],[0 1 1 1-e 1-e 0+e],c3);plot([0 1 1 0 0],[0 0 1 1 0]);disp('weights');
  "IW{2,1}(9,:)'" : Constant  Value=[0.49338485272295429240330122411251068115234375;-1.0311614828162289914104121635318733751773834228515625;-0.85607583530361364143601576870423741638660430908203125;0.336813299768164930991787286984617821872234344482421875;-1.396165686794275995197267548064701259136199951171875;1.25085888191294625215732594369910657405853271484375;-2.157731034925893798259721734211780130863189697265625;-0.837667537999184919073059063521213829517364501953125]
      mask Display: e = 0.06;c1 = [120 150 230]/255;c2 = ([120 150 230]+0)/383;c3 = ([120 150 230]+128)/383;patch([0 1 1 0],[0 0 1 1],c1);patch([0 1 1 1-e 1-e 0+e],[0 0 1 1-e 0+e 0+e],c2);patch([0 0 1 1-e 0+e 0+e],[0 1 1 1-e 1-e 0+e],c3);plot([0 1 1 0 0],[0 0 1 1 0]);disp('weights');
  "IW{2,1}(90,:)'" : Constant  Value=[-0.464172584786029018832920201020897366106510162353515625;-0.138503710006325941872518114905687980353832244873046875;-0.49935020734956270249682575013139285147190093994140625;1.4171494945304023982401986359036527574062347412109375;-0.67941790448352790132702239134232513606548309326171875;2.08394780070833718355061137117445468902587890625;1.801323394221863605224598359200172126293182373046875;-0.6850116149976113177899605943821370601654052734375]
      mask Display: e = 0.06;c1 = [120 150 230]/255;c2 = ([120 150 230]+0)/383;c3 = ([120 150 230]+128)/383;patch([0 1 1 0],[0 0 1 1],c1);patch([0 1 1 1-e 1-e 0+e],[0 0 1 1-e 0+e 0+e],c2);patch([0 0 1 1-e 0+e 0+e],[0 1 1 1-e 1-e 0+e],c3);plot([0 1 1 0 0],[0 0 1 1 0]);disp('weights');
  "IW{2,1}(900,:)'" : Constant  Value=[-1.0850063439514505692073953468934632837772369384765625;0.7359905327501323757388718149741180241107940673828125;1.705284083996837285468473055516369640827178955078125;0.98036451927058987365626308019272983074188232421875;2.075080431180469364704777035512961447238922119140625;1.005456086601173470995718162157572805881500244140625;0.2426096290379319009300473908297135494649410247802734375;0.06958346796512983323257373058368102647364139556884765625]
      mask Display: e = 0.06;c1 = [120 150 230]/255;c2 = ([120 150 230]+0)/383;c3 = ([120 150 230]+128)/383;patch([0 1 1 0],[0 0 1 1],c1);patch([0 1 1 1-e 1-e 0+e],[0 0 1 1-e 0+e 0+e],c2);patch([0 0 1 1-e 0+e 0+e],[0 1 1 1-e 1-e 0+e],c3);plot([0 1 1 0 0],[0 0 1 1 0]);disp('weights');
  "IW{2,1}(901,:)'" : Constant  Value=[1.1996100181406907925207860898808576166629791259765625;-1.3065840329819220499985021888278424739837646484375;-0.499601757030193771580428574452525936067104339599609375;-1.6872088431528411422988256163080222904682159423828125;1.4796534282517106451138033662573434412479400634765625;-1.05545051248295607138061313889920711517333984375;0.719976050472271200675322688766755163669586181640625;-1.0324537590326610114743743906728923320770263671875]
      mask Display: e = 0.06;c1 = [120 150 230]/255;c2 = ([120 150 230]+0)/383;c3 = ([120 150 230]+128)/383;patch([0 1 1 0],[0 0 1 1],c1);patch([0 1 1 1-e 1-e 0+e],[0 0 1 1-e 0+e 0+e],c2);patch([0 0 1 1-e 0+e 0+e],[0 1 1 1-e 1-e 0+e],c3);plot([0 1 1 0 0],[0 0 1 1 0]);disp('weights');
  "IW{2,1}(902,:)'" : Constant  Value=[0.9539806527356147203278169399709440767765045166015625;-0.9696617190083711701475976951769553124904632568359375;0.677689421889368315277124565909616649150848388671875;-2.306096843798648432510844941134564578533172607421875;1.6020463679186445205004929448477923870086669921875;-0.57204234923638164200809796966495923697948455810546875;0.421184754947928896573472457021125592291355133056640625;0.55619552236762748176346349282539449632167816162109375]
      mask Display: e = 0.06;c1 = [120 150 230]/255;c2 = ([120 150 230]+0)/383;c3 = ([120 150 230]+128)/383;patch([0 1 1 0],[0 0 1 1],c1);patch([0 1 1 1-e 1-e 0+e],[0 0 1 1-e 0+e 0+e],c2);patch([0 0 1 1-e 0+e 0+e],[0 1 1 1-e 1-e 0+e],c3);plot([0 1 1 0 0],[0 0 1 1 0]);disp('weights');
  "IW{2,1}(903,:)'" : Constant  Value=[-1.7245723369964363058670642203651368618011474609375;-1.30766721726220769284054767922498285770416259765625;-0.584934536639650115574795563588850200176239013671875;0.76857363358067376513105273261317051947116851806640625;0.90176784960872946594889754123869352042675018310546875;0.996789599884042587518706568516790866851806640625;1.4884721090852310876329056554823182523250579833984375;1.11219834414299700853234753594733774662017822265625]
      mask Display: e = 0.06;c1 = [120 150 230]/255;c2 = ([120 150 230]+0)/383;c3 = ([120 150 230]+128)/383;patch([0 1 1 0],[0 0 1 1],c1);patch([0 1 1 1-e 1-e 0+e],[0 0 1 1-e 0+e 0+e],c2);patch([0 0 1 1-e 0+e 0+e],[0 1 1 1-e 1-e 0+e],c3);plot([0 1 1 0 0],[0 0 1 1 0]);disp('weights');
  "IW{2,1}(904,:)'" : Constant  Value=[-0.325878123027586230620045171235688030719757080078125;-1.614244268583960195684312566299922764301300048828125;1.8047610022579068100867516477592289447784423828125;-0.276935527505401346548552510284935124218463897705078125;-0.30335413058279436793185368514969013631343841552734375;-1.687965835204991993379053383250720798969268798828125;-1.03604320525690685173003657837398350238800048828125;0.96934514658332726622091968238237313926219940185546875]
      mask Display: e = 0.06;c1 = [120 150 230]/255;c2 = ([120 150 230]+0)/383;c3 = ([120 150 230]+128)/383;patch([0 1 1 0],[0 0 1 1],c1);patch([0 1 1 1-e 1-e 0+e],[0 0 1 1-e 0+e 0+e],c2);patch([0 0 1 1-e 0+e 0+e],[0 1 1 1-e 1-e 0+e],c3);plot([0 1 1 0 0],[0 0 1 1 0]);disp('weights');
  "IW{2,1}(905,:)'" : Constant  Value=[0.07316001651718163911741754645845503546297550201416015625;1.8206348362245659000535624727490358054637908935546875;1.661596012936338073728848030441440641880035400390625;0.7642959965284805701202230920898728072643280029296875;-1.8038360812077625094929089755169115960597991943359375;0.261216610595366771629954882882884703576564788818359375;0.6548029171861398101128770576906390488147735595703125;-0.77633463139016345433418564425664953887462615966796875]
      mask Display: e = 0.06;c1 = [120 150 230]/255;c2 = ([120 150 230]+0)/383;c3 = ([120 150 230]+128)/383;patch([0 1 1 0],[0 0 1 1],c1);patch([0 1 1 1-e 1-e 0+e],[0 0 1 1-e 0+e 0+e],c2);patch([0 0 1 1-e 0+e 0+e],[0 1 1 1-e 1-e 0+e],c3);plot([0 1 1 0 0],[0 0 1 1 0]);disp('weights');
  "IW{2,1}(906,:)'" : Constant  Value=[-0.389500832325247292597936166202998720109462738037109375;-0.471696821831662449486799459918984211981296539306640625;-0.9264028941506279313244931472581811249256134033203125;2.041307660797674117247879621572792530059814453125;0.559193945542288073369263656786642968654632568359375;-0.1870683056256715326437500834799720905721187591552734375;1.2272863077649720509043618221767246723175048828125;1.91884785852920725091053100186400115489959716796875]
      mask Display: e = 0.06;c1 = [120 150 230]/255;c2 = ([120 150 230]+0)/383;c3 = ([120 150 230]+128)/383;patch([0 1 1 0],[0 0 1 1],c1);patch([0 1 1 1-e 1-e 0+e],[0 0 1 1-e 0+e 0+e],c2);patch([0 0 1 1-e 0+e 0+e],[0 1 1 1-e 1-e 0+e],c3);plot([0 1 1 0 0],[0 0 1 1 0]);disp('weights');
  "IW{2,1}(907,:)'" : Constant  Value=[-1.526069662272416582737832868588156998157501220703125;-0.346367910022659597490957139598322100937366485595703125;0.05254087283156301524389419910221477039158344268798828125;1.457423930667856470932974843890406191349029541015625;-0.320649626814305810373895155862555839121341705322265625;0.14763878052431689269496928318403661251068115234375;1.81761884474075241513446599128656089305877685546875;1.8012687811654106706527045389520935714244842529296875]
      mask Display: e = 0.06;c1 = [120 150 230]/255;c2 = ([120 150 230]+0)/383;c3 = ([120 150 230]+128)/383;patch([0 1 1 0],[0 0 1 1],c1);patch([0 1 1 1-e 1-e 0+e],[0 0 1 1-e 0+e 0+e],c2);patch([0 0 1 1-e 0+e 0+e],[0 1 1 1-e 1-e 0+e],c3);plot([0 1 1 0 0],[0 0 1 1 0]);disp('weights');
  "IW{2,1}(908,:)'" : Constant  Value=[0.33117165017828364970142729362123645842075347900390625;-0.321234007807936483569477559285587631165981292724609375;0.77867818880135930559305279530235566198825836181640625;1.84259254018791640561403255560435354709625244140625;-1.33834382410176289113223901949822902679443359375;1.0416274574885349135655587815563194453716278076171875;0.1953216804806753026380050641819252632558345794677734375;-1.9778416880248108622453173666144721210002899169921875]
      mask Display: e = 0.06;c1 = [120 150 230]/255;c2 = ([120 150 230]+0)/383;c3 = ([120 150 230]+128)/383;patch([0 1 1 0],[0 0 1 1],c1);patch([0 1 1 1-e 1-e 0+e],[0 0 1 1-e 0+e 0+e],c2);patch([0 0 1 1-e 0+e 0+e],[0 1 1 1-e 1-e 0+e],c3);plot([0 1 1 0 0],[0 0 1 1 0]);disp('weights');
  "IW{2,1}(909,:)'" : Constant  Value=[0.06570765140451671759702634290079004131257534027099609375;1.6724485246177935859890339997946284711360931396484375;0.9887820102882465267413181209121830761432647705078125;1.558030332498313352829200084670446813106536865234375;-1.214453233042798618868118865066207945346832275390625;0.128937873166003302838333866020548157393932342529296875;-1.440778265635862087634677664027549326419830322265625;-1.1158300797147553407029363370384089648723602294921875]
      mask Display: e = 0.06;c1 = [120 150 230]/255;c2 = ([120 150 230]+0)/383;c3 = ([120 150 230]+128)/383;patch([0 1 1 0],[0 0 1 1],c1);patch([0 1 1 1-e 1-e 0+e],[0 0 1 1-e 0+e 0+e],c2);patch([0 0 1 1-e 0+e 0+e],[0 1 1 1-e 1-e 0+e],c3);plot([0 1 1 0 0],[0 0 1 1 0]);disp('weights');
  "IW{2,1}(91,:)'" : Constant  Value=[-1.4446952752452839607855139547609724104404449462890625;0.884466420898849303711131142335943877696990966796875;-0.034965401281585768711313022549802553839981555938720703125;1.6093542570848970996166826807893812656402587890625;1.91211566058573989579372209846042096614837646484375;-1.248684118821994815107245813123881816864013671875;0.56822740529979298695906209104578010737895965576171875;-0.14515676906152286118611982601578347384929656982421875]
      mask Display: e = 0.06;c1 = [120 150 230]/255;c2 = ([120 150 230]+0)/383;c3 = ([120 150 230]+128)/383;patch([0 1 1 0],[0 0 1 1],c1);patch([0 1 1 1-e 1-e 0+e],[0 0 1 1-e 0+e 0+e],c2);patch([0 0 1 1-e 0+e 0+e],[0 1 1 1-e 1-e 0+e],c3);plot([0 1 1 0 0],[0 0 1 1 0]);disp('weights');
  "IW{2,1}(910,:)'" : Constant  Value=[0.857175190635312223008668297552503645420074462890625;0.82291365359157697678682552577811293303966522216796875;1.0769567408869546998317900943220593035221099853515625;-0.61555553728098555410497283446602523326873779296875;-1.249730228189338543387520985561423003673553466796875;-1.795106815461852800552833286928944289684295654296875;0.661656298552848465277520517702214419841766357421875;-1.6319075012263877244578225145232863724231719970703125]
      mask Display: e = 0.06;c1 = [120 150 230]/255;c2 = ([120 150 230]+0)/383;c3 = ([120 150 230]+128)/383;patch([0 1 1 0],[0 0 1 1],c1);patch([0 1 1 1-e 1-e 0+e],[0 0 1 1-e 0+e 0+e],c2);patch([0 0 1 1-e 0+e 0+e],[0 1 1 1-e 1-e 0+e],c3);plot([0 1 1 0 0],[0 0 1 1 0]);disp('weights');
  "IW{2,1}(911,:)'" : Constant  Value=[1.983887447108017898500520459492690861225128173828125;1.125096056857586734878395873238332569599151611328125;-0.408014142812358870937572419279604218900203704833984375;-0.91113874559961904875393656766391359269618988037109375;-0.47832258175421404899907429353334009647369384765625;-0.0385108450736814933446083841772633604705333709716796875;2.03920947614990755170083502889610826969146728515625;-0.6557900211287692737727184066898189485073089599609375]
      mask Display: e = 0.06;c1 = [120 150 230]/255;c2 = ([120 150 230]+0)/383;c3 = ([120 150 230]+128)/383;patch([0 1 1 0],[0 0 1 1],c1);patch([0 1 1 1-e 1-e 0+e],[0 0 1 1-e 0+e 0+e],c2);patch([0 0 1 1-e 0+e 0+e],[0 1 1 1-e 1-e 0+e],c3);plot([0 1 1 0 0],[0 0 1 1 0]);disp('weights');
  "IW{2,1}(912,:)'" : Constant  Value=[-0.73529146193310690460265277579310350120067596435546875;0.417146113922666705864372715950594283640384674072265625;0.362423805552383349048994887198205105960369110107421875;1.7909096905935033561263480805791914463043212890625;0.221079613113343509400721131896716542541980743408203125;-0.138839264913946769386399182621971704065799713134765625;1.7524808015202044675362458292511291801929473876953125;1.8893941209990245955196996874292381107807159423828125]
      mask Display: e = 0.06;c1 = [120 150 230]/255;c2 = ([120 150 230]+0)/383;c3 = ([120 150 230]+128)/383;patch([0 1 1 0],[0 0 1 1],c1);patch([0 1 1 1-e 1-e 0+e],[0 0 1 1-e 0+e 0+e],c2);patch([0 0 1 1-e 0+e 0+e],[0 1 1 1-e 1-e 0+e],c3);plot([0 1 1 0 0],[0 0 1 1 0]);disp('weights');
  "IW{2,1}(913,:)'" : Constant  Value=[-0.50381431980072044485297055871342308819293975830078125;-0.58894893928702829466459434115677140653133392333984375;-0.5340298182171319130162601140909828245639801025390625;0.43205515583611775465300297582871280610561370849609375;-1.89644918270636342327861711964942514896392822265625;-1.3682591953924541083864596657804213464260101318359375;1.8433597798455629845904013563995249569416046142578125;1.04457624074540067482530503184534609317779541015625]
      mask Display: e = 0.06;c1 = [120 150 230]/255;c2 = ([120 150 230]+0)/383;c3 = ([120 150 230]+128)/383;patch([0 1 1 0],[0 0 1 1],c1);patch([0 1 1 1-e 1-e 0+e],[0 0 1 1-e 0+e 0+e],c2);patch([0 0 1 1-e 0+e 0+e],[0 1 1 1-e 1-e 0+e],c3);plot([0 1 1 0 0],[0 0 1 1 0]);disp('weights');
  "IW{2,1}(914,:)'" : Constant  Value=[1.0592162207767972237348885755636729300022125244140625;0.2183264655431417511355363103575655259191989898681640625;1.7371408394069407510329483557143248617649078369140625;-1.4953066565323542835841408304986543953418731689453125;-0.45401666956225461557750122665311209857463836669921875;1.2378343937748714775892722173011861741542816162109375;-0.3339612302818120159741965835564769804477691650390625;-1.6534088180000361401056352406158111989498138427734375]
      mask Display: e = 0.06;c1 = [120 150 230]/255;c2 = ([120 150 230]+0)/383;c3 = ([120 150 230]+128)/383;patch([0 1 1 0],[0 0 1 1],c1);patch([0 1 1 1-e 1-e 0+e],[0 0 1 1-e 0+e 0+e],c2);patch([0 0 1 1-e 0+e 0+e],[0 1 1 1-e 1-e 0+e],c3);plot([0 1 1 0 0],[0 0 1 1 0]);disp('weights');
  "IW{2,1}(915,:)'" : Constant  Value=[0.630031009982552792081378356670029461383819580078125;-0.31904345069296902170918883712147362530231475830078125;0.09388745316407946794878824903207714669406414031982421875;-0.63916939622412283217300910109770484268665313720703125;1.478226253884487473300168858258984982967376708984375;-1.812226966501352620753095834515988826751708984375;-2.078935540018221228564243574510328471660614013671875;0.5328197585085938658977511295233853161334991455078125]
      mask Display: e = 0.06;c1 = [120 150 230]/255;c2 = ([120 150 230]+0)/383;c3 = ([120 150 230]+128)/383;patch([0 1 1 0],[0 0 1 1],c1);patch([0 1 1 1-e 1-e 0+e],[0 0 1 1-e 0+e 0+e],c2);patch([0 0 1 1-e 0+e 0+e],[0 1 1 1-e 1-e 0+e],c3);plot([0 1 1 0 0],[0 0 1 1 0]);disp('weights');
  "IW{2,1}(916,:)'" : Constant  Value=[1.064618150697558718320578918792307376861572265625;-2.618832120980260302900433089234866201877593994140625;0.01183621458994601159664394884885041392408311367034912109375;-0.6339725532473565738911247535725124180316925048828125;0.74225654090177994870458633158705197274684906005859375;1.3045846863981018781686316287959925830364227294921875;0.477891479519270523379503856631345115602016448974609375;-0.396473396188814664053978731317329220473766326904296875]
      mask Display: e = 0.06;c1 = [120 150 230]/255;c2 = ([120 150 230]+0)/383;c3 = ([120 150 230]+128)/383;patch([0 1 1 0],[0 0 1 1],c1);patch([0 1 1 1-e 1-e 0+e],[0 0 1 1-e 0+e 0+e],c2);patch([0 0 1 1-e 0+e 0+e],[0 1 1 1-e 1-e 0+e],c3);plot([0 1 1 0 0],[0 0 1 1 0]);disp('weights');
